simulink model "untitled"  (R2021a)
settings: Solver=VariableStepAuto  StartTime=0.0  StopTime=2  RelTol=1e-3
undefined symbols (not defined in the file or in its folder): sigbuilder_block
libraries: fuzblock x4
(part 2 of 2)

== matlab function untitled/MATLAB Function1 ==
  data: q input; C output; qd input
% Copyright (C) 2022 All rights reserved.
% Authors:     Seonghyeon Jo <cpsc.seonghyeon@gmail.com>
%
% Date:        Jan, 18, 2022
% 
% -------------------------------------------------
% Sawyer Robot 4-DoF
% get a coriolis matrix.
% -------------------------------------------------
% Equation)
%       c(q, dq)
%
% Input)
%       x   : Joint Position
%       dx  : Joint Velocity
% Output)
%       C  : Coriolis Matrix
%
% the following code has been tested on Matlab 2021a
function C = compute_C_4DOF(q,qd)
q1=q(1);
q2=q(2);
q3=q(3);
q4=q(4);
qd1=qd(1);
qd2=qd(2);
qd3=qd(3);
qd4=qd(4);
t2 = cos(q2);
t3 = sin(q2);
t4 = t3.*6.123233995736766e-17;
t5 = t2.*6.123233995736766e-17;
t6 = cos(q3);
t7 = t3-t5;
t8 = sin(q3);
t9 = t3.*3.749399456654644e-33;
t10 = t5+t9;
t11 = cos(q4);
t12 = t2+t4;
t13 = sin(q4);
t16 = t2.*3.749399456654644e-33;
t14 = t4-t16+3.749399456654644e-33;
t24 = t6.*t12;
t25 = t8.*t14;
t15 = t24-t25;
t17 = t6.*t14.*6.123233995736766e-17;
t18 = t8.*t12.*6.123233995736766e-17;
t19 = t3-t5+t17+t18-2.295845021658468e-49;
t20 = sin(q1);
t21 = cos(q1);
t23 = t21.*6.123233995736766e-17;
t22 = t20-t23;
t26 = t6.*t10.*6.123233995736766e-17;
t28 = t7.*t8.*6.123233995736766e-17;
t27 = t2+t4+t26-t28;
t29 = t6.*t7;
t30 = t8.*t10;
t31 = t29+t30;
t32 = t3.*t20.*6.123233995736766e-17;
t33 = t2.*t22;
t34 = t32+t33;
t35 = t2.*t20.*3.749399456654644e-33;
t40 = t3.*t22.*6.123233995736766e-17;
t36 = t35-t40;
t37 = t2.*t20.*6.123233995736766e-17;
t38 = t2.*(t20-t23);
t39 = t32+t38;
t41 = t6.*t36.*6.123233995736766e-17;
t42 = t6.*t39;
t43 = t8.*t36;
t44 = t42+t43;
t46 = t3.*t22;
t45 = t37-t46;
t47 = t20.*6.123233995736766e-17;
t51 = t3.*t20.*3.749399456654644e-33;
t52 = t2.*t22.*6.123233995736766e-17;
t48 = t21+t47-t51-t52;
t49 = t20.*3.749399456654644e-33;
t50 = t8.*t45.*6.123233995736766e-17;
t82 = t6.*t48.*6.123233995736766e-17;
t53 = t23+t32+t38+t49+t50-t82;
t54 = t6.*t45;
t55 = t8.*t48;
t56 = t54+t55;
t57 = t21+t47;
t58 = t2.*t21.*3.749399456654644e-33;
t68 = t3.*t57.*6.123233995736766e-17;
t59 = t58-t68;
t60 = t3.*t21.*6.123233995736766e-17;
t61 = t2.*t57;
t62 = t60+t61;
t63 = t3.*t21.*3.749399456654644e-33;
t64 = t2.*t57.*6.123233995736766e-17;
t65 = t20-t23+t63+t64;
t66 = t2.*t21.*6.123233995736766e-17;
t69 = t3.*t57;
t67 = t66-t69;
t70 = t8.*t59;
t71 = t6.*t62;
t72 = t70+t71;
t73 = t6.*t59.*6.123233995736766e-17;
t83 = t8.*t62.*6.123233995736766e-17;
t74 = t66-t69+t73-t83;
t75 = t21.*3.749399456654644e-33;
t76 = t6.*t65.*6.123233995736766e-17;
t77 = t8.*t67.*6.123233995736766e-17;
t78 = -t47+t60+t61+t75+t76+t77;
t79 = t6.*t67;
t80 = t7.*t8;
t235 = t8.*t39.*6.123233995736766e-17;
t81 = t37+t41-t46-t235;
t85 = t8.*t65;
t84 = t79-t85;
t86 = t6.*t14;
t87 = t8.*t12;
t88 = t8.*t14.*4.4101e-6;
t89 = t21.*1.925e-1;
t90 = t20.*8.100000000000001e-2;
t91 = t3.*t20.*1.688910400704115e-17;
t92 = t8.*t45.*1.4967e-2;
t93 = t2.*(t20-t23).*2.7582e-1;
t333 = t6.*t45.*1.6044e-4;
t334 = t6.*t48.*1.4967e-2;
t335 = t8.*t48.*1.6044e-4;
t94 = t89+t90+t91+t92+t93-t333-t334-t335;
t95 = t86+t87;
t96 = t2.*3.366880115214081e-34;
t97 = t11.*t15.*2.53401226709415e-4;
t98 = t6.*t14.*8.979785040610579e-2;
t99 = t8.*t12.*8.979785040610579e-2;
t201 = t3.*5.498532503507515e-18;
t202 = t13.*t15.*4.876002456295764e-2;
t203 = t11.*t19.*4.876002456295764e-2;
t204 = t13.*t19.*2.53401226709415e-4;
t100 = t96+t97+t98+t99-t201-t202-t203-t204+1.2623778474605e-66;
t101 = -t4+t16+t86+t87+1.405799628556214e-65;
t102 = t6.*t12.*6.123233995736766e-17;
t104 = t8.*t14.*6.123233995736766e-17;
t103 = t102-t104;
t105 = t21.*8.100000000000001e-2;
t106 = t3.*t21.*1.688910400704115e-17;
t107 = t6.*t65.*1.4967e-2;
t108 = t8.*t65.*1.6044e-4;
t109 = t8.*t67.*1.4967e-2;
t110 = t2.*t57.*2.7582e-1;
t282 = t20.*1.925e-1;
t283 = t6.*t67.*1.6044e-4;
t111 = t105+t106+t107+t108+t109+t110-t282-t283;
t112 = t3.*3.3204e-3;
t113 = t6.*t14.*2.53e-2;
t114 = t6.*t12.*4.4101e-6;
t115 = t8.*t12.*2.53e-2;
t116 = t2.*9.157296440624334e-22;
t117 = t6.*t14.*4.4101e-6;
t118 = t8.*t14.*2.5506e-2;
t119 = t8.*t12.*4.4101e-6;
t253 = t3.*1.4955e-5;
t254 = t6.*t12.*2.5506e-2;
t120 = t116+t117+t118+t119-t253-t254+3.433436229890238e-54;
t121 = -t3+t5+2.295845021658468e-49;
t122 = t13.*t15;
t123 = t11.*t19;
t124 = t122+t123;
t125 = t2.*4.271754237092021e-36;
t126 = t11.*t15.*8.169842925973351e-1;
t127 = t6.*t14.*1.139316919009596e-3;
t128 = t8.*t12.*1.139316919009596e-3;
t209 = t3.*6.976304090397628e-20;
t210 = t13.*t15.*2.53401226709415e-4;
t211 = t11.*t19.*2.53401226709415e-4;
t212 = t13.*t19.*8.169842925973351e-1;
t129 = t125+t126+t127+t128-t209-t210-t211-t212+1.6016513015515e-68;
t130 = t2.*2.881087492837848e-33;
t131 = t11.*t15.*1.139316919009596e-3;
t132 = t6.*t14.*7.684130555159526e-1;
t133 = t8.*t12.*7.684130555159526e-1;
t324 = t3.*4.705172944303244e-17;
t325 = t13.*t15.*8.979785040610579e-2;
t326 = t11.*t19.*8.979785040610579e-2;
t327 = t13.*t19.*1.139316919009596e-3;
t134 = t130+t131+t132+t133-t324-t325-t326-t327+1.080234788022072e-65;
t135 = t6.*t67.*6.123233995736766e-17;
t178 = t8.*t65.*6.123233995736766e-17;
t136 = t135-t178;
t137 = t6.*t65;
t138 = t8.*t67;
t139 = t137+t138;
t140 = t21.*8.100000000000001e-2;
t141 = t3.*t21.*2.449293598294706e-17;
t142 = t11.*t78.*2.152934142846781e-1;
t143 = t13.*t78.*9.274373618014111e-4;
t144 = t6.*t65.*1.097689519141626e-1;
t145 = t13.*(t79-t85).*2.152934142846781e-1;
t146 = t8.*t67.*1.097689519141626e-1;
t147 = t2.*t57.*4.0e-1;
t205 = t20.*1.925e-1;
t206 = t11.*t84.*9.274373618014111e-4;
t148 = t140+t141+t142+t143+t144+t145+t146+t147-t205-t206;
t149 = t8.*t45;
t186 = t6.*t48;
t150 = t149-t186;
t151 = t6.*t45.*6.123233995736766e-17;
t152 = t8.*t48.*6.123233995736766e-17;
t153 = t151+t152;
t154 = t21.*1.925e-1;
t155 = t20.*8.100000000000001e-2;
t156 = t3.*t20.*2.449293598294706e-17;
t157 = t8.*t45.*1.097689519141626e-1;
t158 = t2.*(t20-t23).*4.0e-1;
t159 = t11.*t53.*2.152934142846781e-1;
t160 = t13.*t53.*9.274373618014111e-4;
t161 = t13.*t56.*2.152934142846781e-1;
t207 = t11.*t56.*9.274373618014111e-4;
t208 = t6.*t48.*1.097689519141626e-1;
t162 = t154+t155+t156+t157+t158+t159+t160+t161-t207-t208;
t163 = t11.*t15;
t200 = t13.*t19;
t164 = t163-t200;
t165 = t21.*3.359125e-1;
t166 = t20.*1.41345e-1;
t167 = t3.*t20.*2.94714864922868e-17;
t168 = t8.*t45.*2.6117415e-2;
t169 = t2.*(t20-t23).*4.813059e-1;
t249 = t6.*t45.*2.799678e-4;
t250 = t6.*t48.*2.6117415e-2;
t251 = t8.*t48.*2.799678e-4;
t170 = t165+t166+t167+t168+t169-t249-t250-t251;
t171 = t21.*1.41345e-1;
t172 = t3.*t21.*2.94714864922868e-17;
t173 = t6.*t65.*2.6117415e-2;
t174 = t8.*t65.*2.799678e-4;
t175 = t8.*t67.*2.6117415e-2;
t176 = t2.*t57.*4.813059e-1;
t373 = t20.*3.359125e-1;
t374 = t6.*t67.*2.799678e-4;
t177 = t171+t172+t173+t174+t175+t176-t373-t374;
t179 = t21.*4.46715e-1;
t180 = t3.*t21.*1.350785419459531e-16;
t181 = t11.*t78.*1.18734317978;
t182 = t13.*t78.*5.114817050334782e-3;
t183 = t6.*t65.*6.053757698066069e-1;
t184 = t8.*t67.*6.053757698066069e-1;
t185 = t2.*t57.*2.206;
t187 = t21.*1.0616375;
t188 = t20.*4.46715e-1;
t189 = t3.*t20.*1.350785419459531e-16;
t190 = t8.*t45.*6.053757698066069e-1;
t191 = t2.*(t20-t23).*2.206;
t192 = t11.*t53.*1.18734317978;
t193 = t13.*t53.*5.114817050334782e-3;
t194 = t13.*t56.*1.18734317978;
t198 = t11.*t56.*5.114817050334782e-3;
t199 = t6.*t48.*6.053757698066069e-1;
t195 = t187+t188+t189+t190+t191+t192+t193+t194-t198-t199;
t196 = t13.*(t79-t85).*1.18734317978;
t293 = t20.*1.0616375;
t294 = t11.*t84.*5.114817050334782e-3;
t197 = t179+t180+t181+t182+t183+t184+t185+t196-t293-t294;
t213 = t2.*2.398599999999986e-4;
t214 = t3.*2.2398e-2;
t215 = t213+t214;
t216 = t13.*t27;
t217 = t11.*t31;
t218 = t216+t217;
t219 = t2.*t20.*7.395859701019415e-18;
t220 = t3.*t20.*8.509748831328481e-19;
t221 = t21.*1.42521e-1;
t222 = t20.*8.100000000000001e-2;
t223 = t3.*t20.*1.641700266596984e-18;
t224 = t2.*(t20-t23).*2.6811e-2;
t225 = t3.*(t20-t23).*3.0849e-3;
t1223 = t2.*t20.*1.888956455344835e-19;
t226 = t221+t222+t223+t224+t225-t1223;
t227 = t2.*6.976304090397628e-20;
t228 = t3.*4.271754237092021e-36;
t229 = t11.*t27.*2.53401226709415e-4;
t230 = t13.*t27.*8.169842925973351e-1;
t231 = t11.*t31.*8.169842925973351e-1;
t232 = t7.*t8.*1.139316919009596e-3;
t401 = t13.*t31.*2.53401226709415e-4;
t402 = t6.*t10.*1.139316919009596e-3;
t233 = t227+t228+t229+t230+t231+t232-t401-t402;
t234 = t2.*t20.*1.350785419459531e-16;
t236 = t11.*t44.*5.114817050334782e-3;
t237 = t6.*t36.*6.053757698066069e-1;
t238 = t2.*1.4613e-2;
t239 = t3.*2.398600000000009e-4;
t240 = t238+t239;
t241 = (t240.*(t3-t5))./2.0;
t399 = t2.*2.033158615944436e-19;
t242 = t88+t112+t113-t114+t115-t399-7.623123809914776e-52;
t323 = t6.*t10;
t243 = t80-t323;
t244 = t2.*t20.*1.688910400704115e-17;
t245 = t6.*t39.*1.6044e-4;
t246 = t6.*t36.*1.4967e-2;
t247 = t8.*t36.*1.6044e-4;
t385 = t8.*t39.*1.4967e-2;
t481 = t3.*t22.*2.7582e-1;
t248 = t244+t245+t246+t247-t385-t481;
t252 = (t170.*t248)./2.0;
t255 = (t120.*(t29+t30))./2.0;
t256 = t2.*t20.*1.641700266596984e-18;
t257 = t3.*t20.*1.888956455344835e-19;
t258 = t2.*(t20-t23).*3.0849e-3;
t259 = t256+t257+t258-t3.*t22.*2.6811e-2;
t260 = t21.*6.42057105e-1;
t261 = t20.*3.64905e-1;
t262 = t3.*t20.*7.395859701019415e-18;
t263 = t2.*(t20-t23).*1.20783555e-1;
t264 = t3.*(t20-t23).*1.38974745e-2;
t1228 = t2.*t20.*8.509748831328481e-19;
t265 = t260+t261+t262+t263+t264-t1228;
t266 = (t259.*t265)./2.0;
t267 = t2.*t21.*7.395859701019415e-18;
t268 = t3.*t21.*8.509748831328481e-19;
t269 = t2.*t57.*1.38974745e-2;
t1229 = t3.*t57.*1.20783555e-1;
t270 = t267+t268+t269-t1229;
t271 = t21.*8.100000000000001e-2;
t272 = t3.*t21.*1.641700266596984e-18;
t273 = t2.*t57.*2.6811e-2;
t274 = t3.*t57.*3.0849e-3;
t1230 = t20.*1.42521e-1;
t1231 = t2.*t21.*1.888956455344835e-19;
t275 = t271+t272+t273+t274-t1230-t1231;
t276 = (t270.*t275)./2.0;
t277 = t2.*t21.*2.94714864922868e-17;
t278 = t6.*t59.*2.6117415e-2;
t279 = t8.*t59.*2.799678e-4;
t280 = t6.*t62.*2.799678e-4;
t1232 = t8.*t62.*2.6117415e-2;
t1233 = t3.*t57.*4.813059e-1;
t281 = t277+t278+t279+t280-t1232-t1233;
t284 = (t111.*t281)./2.0;
t285 = t11.*t27;
t423 = t13.*t31;
t286 = t285-t423;
t287 = t2.*t21.*2.449293598294706e-17;
t288 = t6.*t59.*1.097689519141626e-1;
t289 = t13.*t74.*9.274373618014111e-4;
t290 = t11.*t72.*9.274373618014111e-4;
t291 = t11.*t74.*2.152934142846781e-1;
t389 = t13.*t72.*2.152934142846781e-1;
t390 = t8.*t62.*1.097689519141626e-1;
t469 = t3.*t57.*4.0e-1;
t292 = t287+t288+t289+t290+t291-t389-t390-t469;
t295 = t2.*t21.*1.641700266596984e-18;
t296 = t3.*t21.*1.888956455344835e-19;
t297 = t2.*t57.*3.0849e-3;
t1235 = t3.*t57.*2.6811e-2;
t298 = t295+t296+t297-t1235;
t299 = t21.*3.64905e-1;
t300 = t3.*t21.*7.395859701019415e-18;
t301 = t2.*t57.*1.20783555e-1;
t302 = t3.*t57.*1.38974745e-2;
t1236 = t20.*6.42057105e-1;
t1237 = t2.*t21.*8.509748831328481e-19;
t303 = t299+t300+t301+t302-t1236-t1237;
t304 = (t298.*t303)./2.0;
t305 = t3.*3.4179e-3;
t306 = t6.*t14.*3.3204e-3;
t307 = t6.*t12.*1.4955e-5;
t308 = t8.*t12.*3.3204e-3;
t457 = t2.*2.092860147402869e-19;
t458 = t8.*t14.*1.4955e-5;
t309 = t305+t306+t307+t308-t457-t458-7.846968699526477e-52;
t310 = (t12.*t309)./2.0;
t311 = t2.*4.705172944303244e-17;
t312 = t3.*2.881087492837848e-33;
t313 = t11.*t27.*8.979785040610579e-2;
t314 = t13.*t27.*1.139316919009596e-3;
t315 = t11.*t31.*1.139316919009596e-3;
t316 = t7.*t8.*7.684130555159526e-1;
t470 = t13.*t31.*8.979785040610579e-2;
t471 = t6.*t10.*7.684130555159526e-1;
t317 = t311+t312+t313+t314+t315+t316-t470-t471;
t318 = t2.*1.4955e-5;
t319 = t3.*9.157296440624334e-22;
t320 = t8.*(t3-t5).*4.4101e-6;
t472 = t6.*t7.*2.5506e-2;
t473 = t6.*t10.*4.4101e-6;
t474 = t8.*t10.*2.5506e-2;
t321 = t318+t319+t320-t472-t473-t474;
t322 = (t15.*t321)./2.0;
t328 = t2.*t20.*2.94714864922868e-17;
t329 = t6.*t39.*2.799678e-4;
t330 = t6.*t36.*2.6117415e-2;
t331 = t8.*t36.*2.799678e-4;
t332 = t328+t329+t330+t331-t3.*t22.*4.813059e-1-t8.*t39.*2.6117415e-2;
t336 = (t94.*t332)./2.0;
t337 = t2.*2.398600000000009e-4;
t1238 = t3.*1.4613e-2;
t338 = t337-t1238+2.282446919238515e-35;
t339 = t2.*5.498532503507515e-18;
t340 = t3.*3.366880115214081e-34;
t341 = t11.*t27.*4.876002456295764e-2;
t342 = t13.*t27.*2.53401226709415e-4;
t343 = t8.*(t3-t5).*8.979785040610579e-2;
t344 = t11.*(t29+t30).*2.53401226709415e-4;
t494 = t13.*t31.*4.876002456295764e-2;
t495 = t6.*t10.*8.979785040610579e-2;
t345 = t339+t340+t341+t342+t343+t344-t494-t495;
t346 = (t124.*t345)./2.0;
t347 = t2.*t20.*2.449293598294706e-17;
t348 = t11.*t81.*2.152934142846781e-1;
t349 = t11.*t44.*9.274373618014111e-4;
t350 = t13.*t81.*9.274373618014111e-4;
t351 = t6.*t36.*1.097689519141626e-1;
t430 = t8.*t39.*1.097689519141626e-1;
t431 = t3.*t22.*4.0e-1;
t432 = t13.*t44.*2.152934142846781e-1;
t352 = t347+t348+t349+t350+t351-t430-t431-t432;
t353 = (t195.*t352)./2.0;
t354 = t2.*t21.*1.350785419459531e-16;
t355 = t6.*t59.*6.053757698066069e-1;
t356 = t13.*t74.*5.114817050334782e-3;
t357 = t11.*t72.*5.114817050334782e-3;
t358 = t11.*t74.*1.18734317978;
t1243 = t13.*t72.*1.18734317978;
t1244 = t8.*t62.*6.053757698066069e-1;
t1245 = t3.*t57.*2.206;
t359 = t354+t355+t356+t357+t358-t1243-t1244-t1245;
t360 = (t148.*t359)./2.0;
t361 = t2.*3.3204e-3;
t362 = t3.*2.033158615944436e-19;
t363 = t6.*(t3-t5).*4.4101e-6;
t364 = t6.*t10.*2.53e-2;
t365 = t8.*t10.*4.4101e-6;
t515 = t7.*t8.*2.53e-2;
t366 = t361+t362+t363+t364+t365-t515;
t367 = (t95.*t366)./2.0;
t368 = t2.*t21.*1.688910400704115e-17;
t369 = t6.*t59.*1.4967e-2;
t370 = t8.*t59.*1.6044e-4;
t371 = t6.*t62.*1.6044e-4;
t451 = t8.*t62.*1.4967e-2;
t528 = t3.*t57.*2.7582e-1;
t372 = t368+t369+t370+t371-t451-t528;
t375 = (t177.*t372)./2.0;
t376 = t2.*3.4179e-3;
t377 = t3.*2.092860147402869e-19;
t378 = t6.*t10.*3.3204e-3;
t521 = t6.*t7.*1.4955e-5;
t522 = t7.*t8.*3.3204e-3;
t523 = t8.*t10.*1.4955e-5;
t379 = t376+t377+t378-t521-t522-t523;
t380 = t2.*2.2398e-2;
t1246 = t3.*2.398599999999986e-4;
t381 = t380-t1246+1.100898668462937e-36;
t382 = t2.*t22.*1.38974745e-2;
t383 = t219+t220+t382-t3.*t22.*1.20783555e-1;
t384 = (t226.*t383)./2.0;
t386 = t6.*t14.*2.5506e-2;
t387 = t8.*t12.*2.5506e-2;
t388 = -t88+t114+t386+t387;
t391 = t13.*t95;
t742 = t11.*t103;
t392 = t391-t742;
t393 = (t100.*t392)./2.0;
t394 = t11.*t95.*1.139316919009596e-3;
t395 = t11.*t103.*8.979785040610579e-2;
t396 = t13.*t103.*1.139316919009596e-3;
t397 = t8.*t14.*7.684130555159526e-1;
t743 = t13.*t95.*8.979785040610579e-2;
t744 = t6.*t12.*7.684130555159526e-1;
t398 = t394+t395+t396+t397-t743-t744;
t400 = (t15.*t242)./2.0;
t403 = t11.*t136.*2.152934142846781e-1;
t404 = t13.*t136.*9.274373618014111e-4;
t405 = t11.*t139.*9.274373618014111e-4;
t406 = t6.*t67.*1.097689519141626e-1;
t407 = t13.*t15.*2.152934142846781e-1;
t408 = t11.*t19.*2.152934142846781e-1;
t409 = t13.*t19.*9.274373618014111e-4;
t410 = t6.*t14.*1.097689519141626e-1;
t411 = t8.*t12.*1.097689519141626e-1;
t412 = (t95.*t120)./2.0;
t413 = t6.*t65.*1.6044e-4;
t414 = t6.*t67.*1.4967e-2;
t415 = t8.*t67.*1.6044e-4;
t854 = t8.*t65.*1.4967e-2;
t416 = t413+t414+t415-t854;
t417 = t6.*t14.*1.4967e-2;
t418 = t8.*t14.*1.6044e-4;
t419 = t8.*t12.*1.4967e-2;
t420 = t6.*t12.*2.53e-2;
t863 = t8.*t14.*2.53e-2;
t421 = t117+t119+t420-t863;
t422 = (t95.*t421)./2.0;
t424 = t11.*(t29+t30);
t425 = t216+t424;
t426 = t5+t9+t80-t323;
t427 = t23+t32+t38+t49;
t428 = t3.*2.6e-1;
t463 = t2.*1.592040838891559e-17;
t464 = t11.*t15.*9.274373618014111e-4;
t429 = t407+t408+t409+t410+t411+t428-t463-t464-5.969197056312016e-50;
t433 = t6.*t14.*1.4955e-5;
t434 = t8.*t14.*3.3204e-3;
t435 = t8.*t12.*1.4955e-5;
t884 = t6.*t12.*3.3204e-3;
t436 = t433+t434+t435-t884;
t437 = (t121.*t436)./2.0;
t438 = t11.*t95.*2.53401226709415e-4;
t439 = t11.*t103.*4.876002456295764e-2;
t440 = t13.*t103.*2.53401226709415e-4;
t441 = t8.*t14.*8.979785040610579e-2;
t745 = t13.*t95.*4.876002456295764e-2;
t746 = t6.*t12.*8.979785040610579e-2;
t442 = t438+t439+t440+t441-t745-t746;
t443 = (t124.*t442)./2.0;
t444 = -t47+t60+t61+t75;
t445 = t2.*1.3582e-1;
t446 = t3.*8.316576413009676e-18;
t447 = t6.*t10.*1.4967e-2;
t448 = t8.*t10.*1.6044e-4;
t449 = t3.*1.3582e-1;
t476 = t2.*8.316576413009676e-18;
t477 = t6.*t12.*1.6044e-4;
t450 = t417+t418+t419+t449-t476-t477-3.118216708416531e-50;
t452 = t6.*t7.*1.6044e-4;
t835 = t7.*t8.*1.4967e-2;
t453 = t445+t446+t447+t448+t452-t835;
t454 = t11.*t95;
t455 = t13.*t103;
t456 = t454+t455;
t459 = t6.*t14.*1.6044e-4;
t460 = t6.*t12.*1.4967e-2;
t461 = t8.*t12.*1.6044e-4;
t849 = t8.*t14.*1.4967e-2;
t462 = t459+t460+t461-t849;
t465 = t21.*9.748438587302075e-34;
t466 = t3.*t21.*1.592040838891559e-17;
t467 = t2.*t57.*2.6e-1;
t709 = t20.*1.592040838891559e-17;
t468 = t142+t143+t144+t145+t146-t206+t465+t466+t467-t709;
t475 = (t15.*t134)./2.0;
t478 = t21.*8.316576413009676e-18;
t479 = t20.*5.092434342028338e-34;
t480 = t3.*t20.*8.316576413009676e-18;
t482 = t2.*t22.*1.3582e-1;
t483 = t92-t333-t334-t335+t478+t479+t480+t482;
t484 = t11.*t95.*8.169842925973351e-1;
t485 = t11.*t103.*2.53401226709415e-4;
t486 = t13.*t103.*8.169842925973351e-1;
t487 = t8.*t14.*1.139316919009596e-3;
t747 = t13.*t95.*2.53401226709415e-4;
t748 = t6.*t12.*1.139316919009596e-3;
t488 = t484+t485+t486+t487-t747-t748;
t489 = t6.*t45.*1.4967e-2;
t490 = t8.*t45.*1.6044e-4;
t491 = t8.*t48.*1.4967e-2;
t492 = t489+t490+t491-t6.*t48.*1.6044e-4;
t493 = t3.*2.7582e-1;
t496 = t13.*t153.*9.274373618014111e-4;
t497 = t6.*t45.*1.097689519141626e-1;
t498 = t11.*t150.*9.274373618014111e-4;
t499 = t8.*t48.*1.097689519141626e-1;
t500 = t11.*t153.*2.152934142846781e-1;
t501 = t496+t497+t498+t499+t500-t13.*t150.*2.152934142846781e-1;
t502 = t3.*4.0e-1;
t503 = t2.*2.6e-1;
t504 = t3.*1.592040838891559e-17;
t505 = t11.*t27.*2.152934142846781e-1;
t506 = t13.*t27.*9.274373618014111e-4;
t507 = t6.*t10.*1.097689519141626e-1;
t508 = t21.*1.592040838891559e-17;
t509 = t20.*9.748438587302075e-34;
t510 = t3.*t20.*1.592040838891559e-17;
t511 = t2.*t22.*2.6e-1;
t512 = t157+t159+t160+t161-t207-t208+t508+t509+t510+t511;
t513 = t11.*t31.*9.274373618014111e-4;
t594 = t13.*t31.*2.152934142846781e-1;
t845 = t7.*t8.*1.097689519141626e-1;
t514 = t503+t504+t505+t506+t507+t513-t594-t845;
t516 = t11.*t95.*9.274373618014111e-4;
t517 = t11.*t103.*2.152934142846781e-1;
t518 = t13.*t103.*9.274373618014111e-4;
t519 = t6.*t12.*1.097689519141626e-1;
t704 = t13.*t95.*2.152934142846781e-1;
t886 = t8.*t14.*1.097689519141626e-1;
t520 = t516+t517+t518+t519-t704-t886;
t524 = t21.*5.092434342028338e-34;
t525 = t3.*t21.*8.316576413009676e-18;
t526 = t2.*t57.*1.3582e-1;
t900 = t20.*8.316576413009676e-18;
t527 = t107+t108+t109-t283+t524+t525+t526-t900;
t529 = t8.*(t3-t5);
t530 = t5+t9-t323+t529;
t531 = t2.*t20.*4.271754237092021e-36;
t532 = t8.*t39.*1.139316919009596e-3;
t533 = t11.*t81.*2.53401226709415e-4;
t534 = t11.*t44.*8.169842925973351e-1;
t535 = t13.*t81.*8.169842925973351e-1;
t536 = t531+t532+t533+t534+t535-t3.*t22.*6.976304090397628e-20-t6.*t36.*1.139316919009596e-3-t13.*t44.*2.53401226709415e-4;
t537 = t21.*3.366880115214081e-34;
t538 = t20.*2.061619478104898e-50;
t539 = t3.*t20.*3.366880115214081e-34;
t540 = t2.*(t20-t23).*5.498532503507515e-18;
t541 = t11.*t53.*4.876002456295764e-2;
t542 = t13.*t53.*2.53401226709415e-4;
t543 = t13.*t56.*4.876002456295764e-2;
t544 = t6.*t48.*8.979785040610579e-2;
t685 = t8.*t45.*8.979785040610579e-2;
t686 = t11.*t56.*2.53401226709415e-4;
t545 = t537+t538+t539+t540+t541+t542+t543+t544-t685-t686;
t546 = t286.*t545;
t547 = t21.*4.271754237092021e-36;
t548 = t20.*2.615695076599444e-52;
t549 = t3.*t20.*4.271754237092021e-36;
t550 = t2.*(t20-t23).*6.976304090397628e-20;
t551 = t11.*t53.*2.53401226709415e-4;
t552 = t13.*t53.*8.169842925973351e-1;
t553 = t13.*t56.*2.53401226709415e-4;
t554 = t6.*t48.*1.139316919009596e-3;
t687 = t8.*t45.*1.139316919009596e-3;
t688 = t11.*t56.*8.169842925973351e-1;
t555 = t547+t548+t549+t550+t551+t552+t553+t554-t687-t688;
t556 = t425.*t555;
t557 = t21.*2.881087492837848e-33;
t558 = t20.*1.764157288083672e-49;
t559 = t3.*t20.*2.881087492837848e-33;
t560 = t2.*(t20-t23).*4.705172944303244e-17;
t561 = t11.*t53.*8.979785040610579e-2;
t562 = t13.*t53.*1.139316919009596e-3;
t563 = t13.*t56.*8.979785040610579e-2;
t564 = t6.*t48.*7.684130555159526e-1;
t683 = t8.*t45.*7.684130555159526e-1;
t684 = t11.*t56.*1.139316919009596e-3;
t565 = t557+t558+t559+t560+t561+t562+t563+t564-t683-t684;
t566 = t530.*t565;
t567 = t2.*t20.*2.881087492837848e-33;
t568 = t8.*t39.*7.684130555159526e-1;
t569 = t11.*t81.*8.979785040610579e-2;
t570 = t11.*t44.*1.139316919009596e-3;
t571 = t13.*t81.*1.139316919009596e-3;
t572 = t567+t568+t569+t570+t571-t3.*t22.*4.705172944303244e-17-t6.*t36.*7.684130555159526e-1-t13.*t44.*8.979785040610579e-2;
t573 = t2.*t20.*3.366880115214081e-34;
t574 = t8.*t39.*8.979785040610579e-2;
t575 = t11.*t81.*4.876002456295764e-2;
t576 = t11.*t44.*2.53401226709415e-4;
t577 = t13.*t81.*2.53401226709415e-4;
t578 = t573+t574+t575+t576+t577-t3.*t22.*5.498532503507515e-18-t6.*t36.*8.979785040610579e-2-t13.*t44.*4.876002456295764e-2;
t579 = t124.*t578;
t580 = t546+t556+t566+t579-t101.*t572-t164.*t536;
t581 = t11.*t78.*9.274373618014111e-4;
t582 = t11.*t84.*2.152934142846781e-1;
t583 = t13.*t84.*9.274373618014111e-4;
t584 = t21.*1.804275904458619e-49;
t585 = t3.*t21.*5.06463411777858e-49;
t701 = t2.*2.449293598294706e-17;
t586 = t407+t408+t409+t410+t411-t464+t502-t701-5.342894225732869e-34;
t587 = t11.*t78.*4.451823873129729e-33;
t588 = t13.*t78.*1.917749226941314e-35;
t589 = t6.*t65.*2.269795582384779e-33;
t590 = t13.*(t79-t85).*4.451823873129729e-33;
t591 = t8.*t67.*2.269795582384779e-33;
t592 = t2.*t57.*8.271175201380145e-33;
t712 = t13.*t78.*2.152934142846781e-1;
t593 = t581+t582+t583-t712;
t595 = t11.*t15.*8.979785040610579e-2;
t596 = t13.*t15.*1.139316919009596e-3;
t597 = t11.*t19.*1.139316919009596e-3;
t749 = t13.*t19.*8.979785040610579e-2;
t598 = t595+t596+t597-t749;
t599 = t20.*2.295845021658468e-49;
t600 = t2.*2.540928714850161e-34;
t601 = t6.*t14.*6.776895191416263e-2;
t602 = t8.*t12.*6.776895191416263e-2;
t641 = t3.*4.149651502162508e-18;
t603 = t407+t408+t409-t464+t600+t601+t602-t641+9.526956742857376e-67;
t604 = t21.*2.540928714850161e-34;
t605 = t20.*1.555870108751424e-50;
t606 = t3.*t20.*2.540928714850161e-34;
t607 = t2.*(t20-t23).*4.149651502162508e-18;
t608 = t6.*t48.*6.776895191416263e-2;
t609 = -t159-t160-t161+t207+t604+t605+t606+t607+t608-t8.*t45.*6.776895191416263e-2;
t610 = t51+t52+t75-t149+t186+t599;
t611 = t13.*t15.*8.169842925973351e-1;
t612 = t11.*t19.*8.169842925973351e-1;
t613 = t97-t204+t611+t612;
t614 = t21.*2.061619478104898e-50;
t615 = t3.*t21.*3.366880115214081e-34;
t616 = t11.*t78.*4.876002456295764e-2;
t617 = t13.*t78.*2.53401226709415e-4;
t618 = t2.*t57.*5.498532503507515e-18;
t619 = t13.*t84.*4.876002456295764e-2;
t668 = t20.*3.366880115214081e-34;
t669 = t6.*t65.*8.979785040610579e-2;
t670 = t11.*t84.*2.53401226709415e-4;
t671 = t8.*t67.*8.979785040610579e-2;
t620 = t614+t615+t616+t617+t618+t619-t668-t669-t670-t671;
t621 = t21.*2.615695076599444e-52;
t622 = t3.*t21.*4.271754237092021e-36;
t623 = t11.*t78.*2.53401226709415e-4;
t624 = t13.*t78.*8.169842925973351e-1;
t625 = t2.*t57.*6.976304090397628e-20;
t626 = t21.*1.764157288083672e-49;
t627 = t3.*t21.*2.881087492837848e-33;
t628 = t11.*t78.*8.979785040610579e-2;
t629 = t13.*t78.*1.139316919009596e-3;
t630 = t2.*t57.*4.705172944303244e-17;
t631 = t8.*(t3-t5).*1.139316919009596e-3;
t632 = t11.*(t29+t30).*8.169842925973351e-1;
t633 = t227+t228+t229+t230-t401-t402+t631+t632;
t634 = t8.*(t3-t5).*7.684130555159526e-1;
t635 = t11.*(t29+t30).*1.139316919009596e-3;
t636 = t311+t312+t313+t314-t470-t471+t634+t635;
t637 = t11.*t15.*2.152934142846781e-1;
t638 = t13.*t15.*9.274373618014111e-4;
t639 = t11.*t19.*9.274373618014111e-4;
t720 = t13.*t19.*2.152934142846781e-1;
t640 = t637+t638+t639-t720;
t642 = t21.*2.295845021658468e-49;
t643 = t2.*4.149651502162508e-18;
t644 = t3.*2.540928714850161e-34;
t645 = t6.*t10.*6.776895191416263e-2;
t646 = t49-t63-t64+t137+t138-t642;
t1187 = t7.*t8.*6.776895191416263e-2;
t647 = t505+t506+t513-t594-t643-t644+t645-t1187;
t648 = t20.*2.540928714850161e-34;
t649 = t6.*t65.*6.776895191416263e-2;
t650 = t8.*t67.*6.776895191416263e-2;
t705 = t21.*1.555870108751424e-50;
t706 = t3.*t21.*2.540928714850161e-34;
t707 = t2.*t57.*4.149651502162508e-18;
t651 = t142+t143+t145-t206+t648+t649+t650-t705-t706-t707;
t652 = t11.*t15.*4.876002456295764e-2;
t821 = t13.*t19.*4.876002456295764e-2;
t653 = t210+t211+t652-t821;
t654 = (t124.*t653)./2.0;
t655 = t2.*t21.*3.366880115214081e-34;
t656 = t13.*t74.*2.53401226709415e-4;
t657 = t11.*t72.*2.53401226709415e-4;
t658 = t8.*t62.*8.979785040610579e-2;
t659 = t11.*t74.*4.876002456295764e-2;
t864 = t6.*t59.*8.979785040610579e-2;
t865 = t13.*t72.*4.876002456295764e-2;
t866 = t3.*t57.*5.498532503507515e-18;
t660 = t655+t656+t657+t658+t659-t864-t865-t866;
t661 = t124.*t660;
t662 = t2.*t21.*4.271754237092021e-36;
t663 = t13.*t74.*8.169842925973351e-1;
t664 = t11.*t72.*8.169842925973351e-1;
t665 = t8.*t62.*1.139316919009596e-3;
t666 = t11.*t74.*2.53401226709415e-4;
t867 = t6.*t59.*1.139316919009596e-3;
t868 = t13.*t72.*2.53401226709415e-4;
t869 = t3.*t57.*6.976304090397628e-20;
t667 = t662+t663+t664+t665+t666-t867-t868-t869;
t672 = t13.*(t79-t85).*2.53401226709415e-4;
t715 = t20.*4.271754237092021e-36;
t716 = t6.*t65.*1.139316919009596e-3;
t717 = t11.*t84.*8.169842925973351e-1;
t718 = t8.*t67.*1.139316919009596e-3;
t673 = t621+t622+t623+t624+t625+t672-t715-t716-t717-t718;
t674 = t13.*(t79-t85).*8.979785040610579e-2;
t737 = t20.*2.881087492837848e-33;
t738 = t6.*t65.*7.684130555159526e-1;
t739 = t11.*t84.*1.139316919009596e-3;
t740 = t8.*t67.*7.684130555159526e-1;
t675 = t626+t627+t628+t629+t630+t674-t737-t738-t739-t740;
t676 = t2.*t21.*2.881087492837848e-33;
t677 = t13.*t74.*1.139316919009596e-3;
t678 = t11.*t72.*1.139316919009596e-3;
t679 = t8.*t62.*7.684130555159526e-1;
t680 = t11.*t74.*8.979785040610579e-2;
t872 = t6.*t59.*7.684130555159526e-1;
t873 = t13.*t72.*8.979785040610579e-2;
t874 = t3.*t57.*4.705172944303244e-17;
t681 = t676+t677+t678+t679+t680-t872-t873-t874;
t682 = t286.*t620;
t689 = t11.*t53.*9.274373618014111e-4;
t690 = t11.*t56.*2.152934142846781e-1;
t691 = t13.*t56.*9.274373618014111e-4;
t692 = t689+t690+t691-t13.*t53.*2.152934142846781e-1;
t693 = t21.*2.946606165491677e-33;
t694 = t20.*1.804275904458619e-49;
t695 = t3.*t20.*5.06463411777858e-49;
t696 = t8.*t45.*2.269795582384779e-33;
t697 = t2.*(t20-t23).*8.271175201380145e-33;
t698 = t11.*t53.*4.451823873129729e-33;
t699 = t13.*t53.*1.917749226941314e-35;
t700 = t13.*t56.*4.451823873129729e-33;
t702 = t57.*t586.*5.515;
t703 = t693+t694+t695+t696+t697+t698+t699+t700+t702-t6.*t48.*2.269795582384779e-33-t11.*t56.*1.917749226941314e-35;
t708 = t429.*t444.*5.515;
t710 = t121.*t468.*5.515;
t711 = t708+t710;
t713 = t101.*t651.*5.515;
t1063 = t603.*t646.*5.515;
t714 = t713-t1063;
t719 = t13.*t84.*2.53401226709415e-4;
t721 = t2.*(t20-t23).*6.123233995736766e-17;
t722 = t51+t75-t149+t186+t599+t721;
t723 = t11.*t53;
t724 = t13.*t56;
t725 = t723+t724;
t726 = t13.*t53;
t727 = -t20+t23;
t728 = t3.*t727;
t729 = t37+t728;
t730 = t2.*t727.*6.123233995736766e-17;
t731 = t21+t47-t51+t730;
t732 = t6.*t729;
t733 = t8.*t731;
t734 = t732+t733;
t735 = t8.*t729.*6.123233995736766e-17;
t752 = t2.*t727;
t753 = t6.*t731.*6.123233995736766e-17;
t736 = t23+t32+t49+t735-t752-t753;
t741 = t726-t11.*t56;
t750 = t6.*t731;
t754 = t8.*t729;
t751 = t51+t75+t599-t730+t750-t754;
t755 = t6.*t729.*6.123233995736766e-17;
t756 = t8.*t731.*6.123233995736766e-17;
t757 = t755+t756;
t758 = t750-t754;
t759 = t11.*t734.*9.274373618014111e-4;
t760 = t11.*t736;
t761 = t13.*t734;
t762 = t760+t761;
t763 = t13.*(t79-t85).*4.876002456295764e-2;
t764 = t614+t615+t616+t617+t618-t668-t669-t670-t671+t763;
t765 = t11.*t734;
t797 = t13.*t736;
t766 = t765-t797;
t767 = t675.*t751;
t768 = t11.*t736.*8.979785040610579e-2;
t769 = t13.*t736.*1.139316919009596e-3;
t770 = t13.*t734.*8.979785040610579e-2;
t771 = t6.*t731.*7.684130555159526e-1;
t790 = t8.*t729.*7.684130555159526e-1;
t791 = t2.*t727.*4.705172944303244e-17;
t792 = t11.*t734.*1.139316919009596e-3;
t772 = t557+t558+t559+t768+t769+t770+t771-t790-t791-t792;
t773 = t11.*t78;
t774 = t13.*(t79-t85);
t775 = t773+t774;
t776 = t11.*t736.*4.876002456295764e-2;
t777 = t13.*t736.*2.53401226709415e-4;
t778 = t13.*t734.*4.876002456295764e-2;
t779 = t6.*t731.*8.979785040610579e-2;
t794 = t8.*t729.*8.979785040610579e-2;
t795 = t2.*t727.*5.498532503507515e-18;
t796 = t11.*t734.*2.53401226709415e-4;
t780 = t537+t538+t539+t776+t777+t778+t779-t794-t795-t796;
t781 = t775.*t780;
t782 = t13.*t78;
t793 = t11.*t84;
t783 = t782-t793;
t784 = t11.*t736.*2.53401226709415e-4;
t785 = t13.*t736.*8.169842925973351e-1;
t786 = t13.*t734.*2.53401226709415e-4;
t787 = t6.*t731.*1.139316919009596e-3;
t798 = t8.*t729.*1.139316919009596e-3;
t799 = t2.*t727.*6.976304090397628e-20;
t800 = t11.*t734.*8.169842925973351e-1;
t788 = t547+t548+t549+t784+t785+t786+t787-t798-t799-t800;
t789 = t783.*t788;
t801 = t646.*t675;
t802 = t11.*t736.*9.274373618014111e-4;
t803 = t11.*t734.*2.152934142846781e-1;
t804 = t13.*t734.*9.274373618014111e-4;
t1111 = t13.*t736.*2.152934142846781e-1;
t805 = t802+t803+t804-t1111;
t806 = t23+t32+t49-t752;
t807 = t8.*t729.*1.097689519141626e-1;
t808 = t11.*t736.*2.152934142846781e-1;
t809 = t13.*t736.*9.274373618014111e-4;
t810 = t13.*t734.*2.152934142846781e-1;
t811 = t764.*t775;
t812 = t673.*t783;
t813 = -t801+t811+t812;
t819 = t646.*t772;
t814 = t781+t789-t819;
t815 = t751.*t772;
t816 = t762.*t780;
t817 = t762.*t764;
t818 = t129.*t783.*3.749399456654644e-33;
t820 = t100.*t775.*3.749399456654644e-33;
t822 = t6.*t12.*6.776895191416263e-2;
t1058 = t8.*t14.*6.776895191416263e-2;
t823 = t516+t517+t518-t704+t822-t1058;
t824 = t6.*t731.*6.776895191416263e-2;
t825 = t13.*t757.*9.274373618014111e-4;
t826 = t11.*t757.*2.152934142846781e-1;
t830 = t6.*t731.*1.097689519141626e-1;
t888 = t2.*t727.*4.0e-1;
t827 = t154+t155+t156-t759+t807+t808+t809+t810-t830-t888;
t828 = t13.*t758.*2.152934142846781e-1;
t833 = t13.*t139.*2.152934142846781e-1;
t853 = t8.*t65.*1.097689519141626e-1;
t829 = t403+t404+t405+t406-t833-t853;
t1032 = t766.*t788;
t831 = t801-t811-t812+t815+t816-t1032;
t1028 = t673.*t766;
t832 = t767+t781+t789+t817-t819-t1028;
t1107 = t8.*t729.*6.776895191416263e-2;
t1108 = t2.*t727.*4.149651502162508e-18;
t834 = t604+t605+t606+t759-t808-t809-t810+t824-t1107-t1108;
t836 = t2.*t20.*8.316576413009676e-18;
t837 = t32-t752;
t838 = t3.*t727.*6.123233995736766e-17;
t839 = t35+t838;
t840 = t8.*t729.*1.4967e-2;
t841 = t2.*t21.*1.592040838891559e-17;
t1359 = t3.*t57.*2.6e-1;
t842 = t288+t289+t290+t291-t389-t390+t841-t1359;
t843 = t121.*t842.*5.515;
t844 = t67.*t429.*5.515;
t846 = t444.*t514.*5.515;
t1560 = t12.*t468.*5.515;
t847 = t843+t844+t846-t1560;
t848 = t129.*t425.*1.874699728327322e-33;
t850 = t57.*t462.*(3.49e2./2.0e2);
t911 = t6.*t729.*1.6044e-4;
t912 = t6.*t731.*1.4967e-2;
t913 = t8.*t731.*1.6044e-4;
t979 = t2.*t727.*2.7582e-1;
t851 = t89+t90+t91+t840-t911-t912-t913-t979;
t852 = t164.*t633.*1.874699728327322e-33;
t855 = t21.*5.708905626981487e-50;
t856 = t3.*t21.*1.105003754409848e-49;
t857 = t6.*t65.*9.792462161022385e-35;
t858 = t8.*t65.*1.049711117200796e-36;
t919 = t2.*1.688910400704115e-17;
t859 = t417+t418+t419-t477+t493-t919-5.342894225732868e-34;
t860 = t8.*t67.*9.792462161022385e-35;
t861 = t2.*t57.*1.804608079944675e-33;
t862 = t242.*(t80-t323).*1.874699728327322e-33;
t870 = t425.*t673;
t871 = t530.*t675;
t875 = t429.*t806.*5.515;
t968 = t2.*t727.*2.6e-1;
t876 = t508+t509+t510-t759+t807+t808+t809+t810-t830-t968;
t877 = t121.*t876.*5.515;
t878 = t875+t877;
t879 = t6.*t839.*6.123233995736766e-17;
t963 = t8.*t837.*6.123233995736766e-17;
t880 = t37+t728+t879-t963;
t881 = t6.*t837;
t882 = t8.*t839;
t883 = t881+t882;
t885 = t100.*t286.*1.874699728327322e-33;
t887 = t57.*t520.*5.515;
t889 = t21.*9.157296440624334e-22;
t890 = t20.*5.60722688742702e-38;
t891 = t3.*t20.*9.157296440624334e-22;
t892 = t21.*2.033158615944436e-19;
t893 = t20.*1.244950595587608e-35;
t894 = t3.*t20.*2.033158615944436e-19;
t895 = t21.*2.092860147402869e-19;
t896 = t20.*1.281507240289991e-35;
t897 = t3.*t20.*2.092860147402869e-19;
t898 = t2.*t20.*2.033158615944436e-19;
t899 = t67.*t450.*(3.49e2./2.0e2);
t901 = t2.*t21.*8.316576413009676e-18;
t1350 = t3.*t57.*1.3582e-1;
t902 = t369+t370+t371-t451+t901-t1350;
t903 = t121.*t902.*(3.49e2./2.0e2);
t904 = t444.*t453.*(3.49e2./2.0e2);
t1425 = t12.*t527.*(3.49e2./2.0e2);
t905 = t899+t903+t904-t1425;
t906 = t6.*t65.*1.049711117200796e-36;
t907 = t6.*t67.*9.792462161022385e-35;
t908 = t8.*t67.*1.049711117200796e-36;
t909 = t101.*t636.*1.874699728327322e-33;
t910 = t134.*t530.*1.874699728327322e-33;
t914 = t6.*t837.*1.6044e-4;
t915 = t6.*t839.*1.4967e-2;
t916 = t8.*t839.*1.6044e-4;
t917 = t21.*9.323350423903855e-34;
t918 = t20.*5.708905626981487e-50;
t920 = t57.*t859.*(3.49e2./2.0e2);
t921 = t3.*t20.*1.105003754409848e-49;
t922 = t6.*t729.*1.097689519141626e-1;
t923 = t8.*t731.*1.097689519141626e-1;
t924 = t21.*1.244950595587608e-35;
t925 = t3.*t21.*2.033158615944436e-19;
t926 = t6.*t65.*2.53e-2;
t927 = t8.*t65.*4.4101e-6;
t928 = t8.*t67.*2.53e-2;
t929 = t2.*t57.*3.3204e-3;
t1005 = t20.*2.033158615944436e-19;
t1006 = t6.*t67.*4.4101e-6;
t930 = t924+t925+t926+t927+t928+t929-t1005-t1006;
t931 = t6.*t59.*4.4101e-6;
t932 = t8.*t59.*2.5506e-2;
t933 = t6.*t62.*2.5506e-2;
t934 = t3.*t57.*1.4955e-5;
t1523 = t2.*t21.*9.157296440624334e-22;
t1524 = t8.*t62.*4.4101e-6;
t935 = t931+t932+t933+t934-t1523-t1524;
t936 = t21.*1.281507240289991e-35;
t937 = t3.*t21.*2.092860147402869e-19;
t938 = t6.*t65.*3.3204e-3;
t939 = t6.*t67.*1.4955e-5;
t940 = t8.*t67.*3.3204e-3;
t941 = t2.*t57.*3.4179e-3;
t1013 = t20.*2.092860147402869e-19;
t1014 = t8.*t65.*1.4955e-5;
t942 = t936+t937+t938+t939+t940+t941-t1013-t1014;
t943 = t12.*t942;
t944 = t2.*t21.*2.033158615944436e-19;
t945 = t6.*t59.*2.53e-2;
t946 = t8.*t59.*4.4101e-6;
t947 = t6.*t62.*4.4101e-6;
t1526 = t8.*t62.*2.53e-2;
t1527 = t3.*t57.*3.3204e-3;
t948 = t944+t945+t946+t947-t1526-t1527;
t949 = t95.*t948;
t950 = t8.*t59.*1.4955e-5;
t951 = t6.*t62.*1.4955e-5;
t952 = t8.*t62.*3.3204e-3;
t953 = t3.*t57.*3.4179e-3;
t1528 = t2.*t21.*2.092860147402869e-19;
t1529 = t6.*t59.*3.3204e-3;
t954 = t950+t951+t952+t953-t1528-t1529;
t955 = t121.*t954;
t956 = t20.*9.157296440624334e-22;
t957 = t3.*t21.*9.157296440624334e-22;
t958 = t6.*t67.*2.5506e-2;
t959 = t2.*t57.*1.4955e-5;
t997 = t21.*5.60722688742702e-38;
t998 = t6.*t65.*4.4101e-6;
t999 = t8.*t65.*2.5506e-2;
t1000 = t8.*t67.*4.4101e-6;
t960 = -t956+t957+t958+t959+t997-t998-t999-t1000;
t1522 = t243.*t930;
t1525 = t15.*t935;
t1530 = t31.*t960;
t961 = t943+t949+t955-t1522-t1525-t1530;
t962 = t2.*t20.*1.592040838891559e-17;
t964 = t11.*t880.*2.152934142846781e-1;
t965 = t11.*t883.*9.274373618014111e-4;
t966 = t13.*t880.*9.274373618014111e-4;
t967 = t6.*t839.*1.097689519141626e-1;
t969 = t11.*t136.*4.451823873129729e-33;
t970 = t13.*t136.*1.917749226941314e-35;
t971 = t11.*t139.*1.917749226941314e-35;
t972 = t6.*t67.*2.269795582384779e-33;
t973 = t121.*t379.*1.874699728327322e-33;
t974 = t444.*t450.*(3.49e2./2.0e2);
t975 = t121.*t527.*(3.49e2./2.0e2);
t976 = t974+t975;
t995 = t11.*t758.*9.274373618014111e-4;
t977 = t825+t826+t828+t922+t923-t995;
t1322 = t2.*t727.*1.3582e-1;
t978 = t478+t479+t480+t840-t911-t912-t913-t1322;
t980 = t6.*t65.*2.799678e-4;
t981 = t6.*t67.*2.6117415e-2;
t982 = t8.*t67.*2.799678e-4;
t1361 = t8.*t65.*2.6117415e-2;
t983 = t980+t981+t982-t1361;
t984 = (t111.*t983)./2.0;
t985 = t11.*t136.*1.18734317978;
t986 = t13.*t136.*5.114817050334782e-3;
t987 = t11.*t139.*5.114817050334782e-3;
t988 = t6.*t67.*6.053757698066069e-1;
t1351 = t8.*t65.*6.053757698066069e-1;
t1352 = t13.*t139.*1.18734317978;
t2028 = t985+t986+t987+t988-t1351-t1352;
t989 = (t148.*t2028)./2.0;
t990 = t6.*t729.*1.4967e-2;
t991 = t8.*t729.*1.6044e-4;
t992 = t8.*t731.*1.4967e-2;
t1370 = t6.*t731.*1.6044e-4;
t993 = t990+t991+t992-t1370;
t994 = (t177.*t416)./2.0;
t996 = (t197.*t829)./2.0;
t1001 = t6.*t729.*2.5506e-2;
t1002 = t6.*t731.*4.4101e-6;
t1003 = t8.*t731.*2.5506e-2;
t1017 = t8.*t729.*4.4101e-6;
t1018 = t2.*t727.*1.4955e-5;
t1004 = t889+t890+t891+t1001+t1002+t1003-t1017-t1018;
t1007 = t8.*t729.*2.53e-2;
t1019 = t6.*t729.*4.4101e-6;
t1020 = t2.*t727.*3.3204e-3;
t1021 = t6.*t731.*2.53e-2;
t1022 = t8.*t731.*4.4101e-6;
t1008 = t892+t893+t894+t1007-t1019-t1020-t1021-t1022;
t1009 = t6.*t729.*1.4955e-5;
t1010 = t8.*t729.*3.3204e-3;
t1011 = t8.*t731.*1.4955e-5;
t1015 = t2.*t727.*3.4179e-3;
t1016 = t6.*t731.*3.3204e-3;
t1012 = t895+t896+t897+t1009+t1010+t1011-t1015-t1016;
t1023 = t444.*t1012;
t1024 = t1004.*(t79-t85);
t1025 = t139.*t1008;
t1026 = t139.*t930;
t1027 = t444.*t942;
t1029 = t727.*t832;
t1030 = t100.*t762.*3.749399456654644e-33;
t1031 = t134.*t751.*3.749399456654644e-33;
t1033 = t57.*t813;
t1034 = t727.*t813;
t1035 = t57.*t814;
t1038 = t134.*t646.*3.749399456654644e-33;
t1036 = t818+t820+t1034+t1035-t1038;
t1037 = t57.*t832;
t1039 = t242.*(t750-t754).*3.749399456654644e-33;
t1040 = t120.*t734.*3.749399456654644e-33;
t1041 = t734.*t960;
t1042 = t806.*t942;
t1043 = t758.*t1008;
t1044 = t960.*(t79-t85);
t1045 = t1026+t1027+t1044;
t1046 = t1023+t1024+t1025;
t1047 = t815+t816-t1032;
t1048 = t767+t817-t1028;
t1049 = t734.*t1004;
t1050 = t806.*t1012;
t1051 = -t1043+t1049+t1050;
t1053 = t758.*t930;
t1052 = t1041+t1042-t1053;
t1054 = t84.*t960;
t1055 = t84.*t120.*3.749399456654644e-33;
t1056 = t6.*t67.*6.776895191416263e-2;
t1851 = t8.*t65.*6.776895191416263e-2;
t1852 = t403+t404+t405-t833+t1056-t1851;
t1057 = t101.*t1852.*5.515;
t1059 = t15.*t651.*5.515;
t1898 = t84.*t603.*5.515;
t1899 = t646.*t823.*5.515;
t1060 = t1057+t1059-t1898-t1899;
t1061 = (t148.*t1060)./2.0;
t1062 = t100.*t164.*1.874699728327322e-33;
t1064 = t11.*t78.*1.139316919009596e-3;
t1065 = t11.*t84.*8.979785040610579e-2;
t1066 = t13.*t84.*1.139316919009596e-3;
t1824 = t13.*t78.*8.979785040610579e-2;
t1067 = t1064+t1065+t1066-t1824;
t1068 = t11.*t78.*8.169842925973351e-1;
t1069 = t13.*t84.*8.169842925973351e-1;
t1070 = -t617+t670+t1068+t1069;
t1071 = t124.*t673;
t1072 = t11.*t84.*4.876002456295764e-2;
t1826 = t13.*t78.*4.876002456295764e-2;
t1073 = t124.*(t623+t719+t1072-t1826);
t1074 = t100.*t762;
t1075 = t134.*t751;
t1142 = t129.*t766;
t1076 = t1074+t1075-t1142;
t1077 = t121.*t1076;
t1078 = t121.*t593.*5.515;
t1079 = t444.*t640.*5.515;
t1080 = t1078+t1079;
t1081 = t100.*t392;
t1082 = t124.*t442;
t1083 = t15.*t134;
t1829 = t101.*t398;
t1830 = t129.*t456;
t1831 = t164.*t488;
t1084 = t1081+t1082+t1083-t1829-t1830-t1831;
t1085 = (t121.*t1084)./2.0;
t1086 = t101.*t598.*1.874699728327322e-33;
t1087 = t164.*t613.*1.874699728327322e-33;
t1088 = t392.*t764;
t1089 = t11.*t136.*4.876002456295764e-2;
t1090 = t13.*t136.*2.53401226709415e-4;
t1091 = t8.*t65.*8.979785040610579e-2;
t1092 = t11.*t139.*2.53401226709415e-4;
t1859 = t6.*t67.*8.979785040610579e-2;
t1860 = t13.*t139.*4.876002456295764e-2;
t1093 = t1089+t1090+t1091+t1092-t1859-t1860;
t1094 = t11.*t136.*2.53401226709415e-4;
t1095 = t13.*t136.*8.169842925973351e-1;
t1096 = t8.*t65.*1.139316919009596e-3;
t1097 = t11.*t139.*8.169842925973351e-1;
t1862 = t6.*t67.*1.139316919009596e-3;
t1863 = t13.*t139.*2.53401226709415e-4;
t2210 = t1094+t1095+t1096+t1097-t1862-t1863;
t1098 = t164.*t2210;
t1099 = t15.*t675;
t1100 = t11.*t136.*8.979785040610579e-2;
t1101 = t13.*t136.*1.139316919009596e-3;
t1102 = t8.*t65.*7.684130555159526e-1;
t1103 = t11.*t139.*1.139316919009596e-3;
t1864 = t6.*t67.*7.684130555159526e-1;
t1865 = t13.*t139.*8.979785040610579e-2;
t2207 = t1100+t1101+t1102+t1103-t1864-t1865;
t1104 = t101.*t2207;
t1858 = t456.*t673;
t1861 = t124.*t1093;
t1105 = t1088+t1098+t1099+t1104-t1858-t1861;
t1106 = (t444.*t1105)./2.0;
t1109 = t101.*t834.*5.515;
t1188 = t603.*t751.*5.515;
t1110 = t1109-t1188;
t1112 = t124.*t129.*1.874699728327322e-33;
t1113 = t121.*t805.*5.515;
t1114 = t640.*t806.*5.515;
t1115 = t1113+t1114;
t1116 = t129.*t783;
t1117 = t100.*t775;
t1138 = t134.*t646;
t1118 = t1116+t1117-t1138;
t1119 = t121.*t1118;
t1120 = t603.*t734.*5.515;
t1121 = t15.*t834.*5.515;
t1122 = t6.*t729.*6.776895191416263e-2;
t1123 = t8.*t731.*6.776895191416263e-2;
t1124 = t6.*t729.*7.684130555159526e-1;
t1125 = t11.*t758.*1.139316919009596e-3;
t1126 = t8.*t731.*7.684130555159526e-1;
t1900 = t13.*t757.*1.139316919009596e-3;
t1901 = t11.*t757.*8.979785040610579e-2;
t1902 = t13.*t758.*8.979785040610579e-2;
t1127 = t1124+t1125+t1126-t1900-t1901-t1902;
t1128 = t15.*t772;
t1129 = t6.*t729.*8.979785040610579e-2;
t1130 = t11.*t758.*2.53401226709415e-4;
t1131 = t8.*t731.*8.979785040610579e-2;
t1132 = t392.*t780;
t1133 = t6.*t729.*1.139316919009596e-3;
t1134 = t11.*t758.*8.169842925973351e-1;
t1135 = t8.*t731.*1.139316919009596e-3;
t1904 = t13.*t757.*8.169842925973351e-1;
t1905 = t11.*t757.*2.53401226709415e-4;
t1906 = t13.*t758.*2.53401226709415e-4;
t1136 = t1133+t1134+t1135-t1904-t1905-t1906;
t1137 = t444.*t813;
t1139 = t806.*t814;
t1140 = t1119+t1137+t1139;
t1141 = t444.*t1048;
t1143 = t806.*t1047;
t1144 = t1077+t1141+t1143;
t1145 = t444.*t832;
t1146 = t806.*t813;
t1147 = t444.*t1047;
t1148 = t806.*t832;
t2025 = t444.*t831;
t2026 = t806.*t1048;
t1149 = t1119+t1147+t1148-t2025-t2026;
t1150 = (t197.*t593)./2.0;
t1151 = t8.*t729.*6.053757698066069e-1;
t1152 = t11.*t736.*1.18734317978;
t1153 = t13.*t736.*5.114817050334782e-3;
t1154 = t13.*t734.*1.18734317978;
t1240 = t2.*t727.*2.206;
t1241 = t11.*t734.*5.114817050334782e-3;
t1242 = t6.*t731.*6.053757698066069e-1;
t1155 = t187+t188+t189+t1151+t1152+t1153+t1154-t1240-t1241-t1242;
t1156 = t11.*t78.*5.114817050334782e-3;
t1157 = t11.*t84.*1.18734317978;
t1158 = t13.*t84.*5.114817050334782e-3;
t1295 = t13.*t78.*1.18734317978;
t1159 = t1156+t1157+t1158-t1295;
t1160 = (t148.*t1159)./2.0;
t1161 = t8.*t837.*1.139316919009596e-3;
t1162 = t11.*t880.*2.53401226709415e-4;
t1163 = t11.*t883.*8.169842925973351e-1;
t1164 = t3.*t727.*6.976304090397628e-20;
t1165 = t13.*t880.*8.169842925973351e-1;
t1545 = t13.*t883.*2.53401226709415e-4;
t1546 = t6.*t839.*1.139316919009596e-3;
t1166 = t531+t1161+t1162+t1163+t1164+t1165-t1545-t1546;
t1167 = t286.*t780;
t1168 = t425.*t788;
t1169 = t530.*t772;
t1170 = t8.*t837.*7.684130555159526e-1;
t1171 = t11.*t880.*8.979785040610579e-2;
t1172 = t11.*t883.*1.139316919009596e-3;
t1173 = t3.*t727.*4.705172944303244e-17;
t1174 = t13.*t880.*1.139316919009596e-3;
t1548 = t13.*t883.*8.979785040610579e-2;
t1549 = t6.*t839.*7.684130555159526e-1;
t1175 = t567+t1170+t1171+t1172+t1173+t1174-t1548-t1549;
t1176 = t8.*t837.*8.979785040610579e-2;
t1177 = t11.*t880.*4.876002456295764e-2;
t1178 = t11.*t883.*2.53401226709415e-4;
t1179 = t3.*t727.*5.498532503507515e-18;
t1180 = t13.*t880.*2.53401226709415e-4;
t1551 = t13.*t883.*4.876002456295764e-2;
t1552 = t6.*t839.*8.979785040610579e-2;
t1181 = t573+t1176+t1177+t1178+t1179+t1180-t1551-t1552;
t1182 = t124.*t1181;
t1547 = t164.*t1166;
t1550 = t101.*t1175;
t1183 = t1167+t1168+t1169+t1182-t1547-t1550;
t1184 = t57.*t640.*5.515;
t1185 = t586.*t727.*5.515;
t1401 = t20.*2.946606165491677e-33;
t1402 = t11.*t84.*1.917749226941314e-35;
t1186 = t584+t585+t587+t588+t589+t590+t591+t592+t1185-t1401-t1402;
t1189 = t3.*t727.*4.0e-1;
t1222 = t13.*t883.*2.152934142846781e-1;
t1239 = t8.*t837.*1.097689519141626e-1;
t1190 = t347+t964+t965+t966+t967+t1189-t1222-t1239;
t1191 = t164.*t673;
t1192 = t101.*t675;
t1193 = t129.*t425;
t1194 = t164.*t633;
t1195 = t100.*t286;
t1196 = t101.*t636;
t1197 = t134.*t530;
t1270 = t124.*t345;
t1198 = t1193+t1194+t1195+t1196+t1197-t1270;
t1199 = (t121.*t1198)./2.0;
t1200 = t11.*t78.*1.917749226941314e-35;
t1201 = t11.*t84.*4.451823873129729e-33;
t1202 = t13.*t84.*1.917749226941314e-35;
t1203 = t129.*t164;
t1204 = t101.*t134;
t1311 = t100.*t124;
t1205 = t1203+t1204-t1311;
t1206 = (t12.*t1205)./2.0;
t1207 = t8.*t62;
t1306 = t6.*t59;
t1208 = t58-t68+t1207-t1306;
t1209 = t6.*t59.*6.776895191416263e-2;
t1210 = t3.*t57.*4.149651502162508e-18;
t1309 = t2.*t21.*2.540928714850161e-34;
t1310 = t8.*t62.*6.776895191416263e-2;
t1211 = t289+t290+t291-t389+t1209+t1210-t1309-t1310;
t1212 = t11.*(t29+t30).*9.274373618014111e-4;
t1213 = t505+t506-t594-t643-t644+t645-t1187+t1212;
t1214 = t530.*t651.*5.515;
t1215 = t286.*t764;
t1416 = t164.*t667;
t1417 = t101.*t681;
t1216 = t661+t870+t871+t1215-t1416-t1417;
t1217 = t8.*t729.*2.269795582384779e-33;
t1218 = t11.*t736.*4.451823873129729e-33;
t1219 = t13.*t736.*1.917749226941314e-35;
t1220 = t13.*t734.*4.451823873129729e-33;
t1479 = t2.*t727.*8.271175201380145e-33;
t1480 = t11.*t734.*1.917749226941314e-35;
t1481 = t6.*t731.*2.269795582384779e-33;
t1221 = t693+t694+t695+t702+t1217+t1218+t1219+t1220-t1479-t1480-t1481;
t1224 = t3.*t727.*2.7582e-1;
t1357 = t8.*t837.*1.4967e-2;
t1225 = t244+t914+t915+t916+t1224-t1357;
t1226 = t8.*t729.*2.6117415e-2;
t1266 = t6.*t729.*2.799678e-4;
t1267 = t2.*t727.*4.813059e-1;
t1268 = t6.*t731.*2.6117415e-2;
t1269 = t8.*t731.*2.799678e-4;
t1227 = t165+t166+t167+t1226-t1266-t1267-t1268-t1269;
t1234 = (t197.*t292)./2.0;
t1247 = t6.*t837.*2.799678e-4;
t1248 = t3.*t727.*4.813059e-1;
t1249 = t6.*t839.*2.6117415e-2;
t1250 = t8.*t839.*2.799678e-4;
t1323 = t8.*t837.*2.6117415e-2;
t1251 = t328+t1247+t1248+t1249+t1250-t1323;
t1704 = t2.*t727.*1.20783555e-1;
t1705 = t3.*t727.*1.38974745e-2;
t1252 = t260+t261+t262-t1228-t1704-t1705;
t1253 = t3.*t727.*1.20783555e-1;
t1711 = t2.*t727.*1.38974745e-2;
t1254 = t219+t220+t1253-t1711;
t1255 = t2.*3.084900000000001e-3;
t1653 = t3.*2.6811e-2;
t1256 = t1255-t1653+3.468981871291444e-34;
t1257 = t2.*4.0e-1;
t1258 = t3.*2.449293598294706e-17;
t1259 = t505+t506+t507-t594-t845+t1212+t1257+t1258;
t1260 = t11.*t880.*1.18734317978;
t1261 = t11.*t883.*5.114817050334782e-3;
t1262 = t3.*t727.*2.206;
t1263 = t13.*t880.*5.114817050334782e-3;
t1264 = t6.*t839.*6.053757698066069e-1;
t1307 = t8.*t837.*6.053757698066069e-1;
t1308 = t13.*t883.*1.18734317978;
t1265 = t234+t1260+t1261+t1262+t1263+t1264-t1307-t1308;
t1271 = t2.*2.7582e-1;
t1272 = t3.*1.688910400704115e-17;
t1273 = t6.*(t3-t5).*1.6044e-4;
t1274 = t447+t448-t835+t1271+t1272+t1273;
t1275 = t2.*2.6811e-2;
t1276 = t3.*3.084900000000001e-3;
t1277 = t1275+t1276;
t1278 = t11.*t736.*5.114817050334782e-3;
t1279 = t11.*t734.*1.18734317978;
t1280 = t13.*t734.*5.114817050334782e-3;
t1981 = t13.*t736.*1.18734317978;
t1281 = t1278+t1279+t1280-t1981;
t1282 = t21.*5.342894225732869e-34;
t1283 = t20.*3.271579155863317e-50;
t1284 = t3.*t20.*9.18338008663387e-50;
t1285 = t8.*t729.*4.115676486645111e-34;
t1286 = t11.*t736.*8.072210105402954e-34;
t1287 = t13.*t736.*3.477333140419428e-36;
t1288 = t13.*t734.*8.072210105402954e-34;
t1289 = t57.*t586;
t1337 = t2.*t727.*1.499759782661858e-33;
t1338 = t11.*t734.*3.477333140419428e-36;
t1339 = t6.*t731.*4.115676486645111e-34;
t1290 = t1282+t1283+t1284+t1285+t1286+t1287+t1288+t1289-t1337-t1338-t1339;
t1291 = t6.*t839.*6.776895191416263e-2;
t1292 = t8.*t837;
t1294 = t6.*t839;
t1293 = t35+t838+t1292-t1294;
t1296 = t21.*3.271579155863317e-50;
t1297 = t3.*t21.*9.18338008663387e-50;
t1298 = t586.*t727;
t1299 = t11.*t78.*8.072210105402954e-34;
t1300 = t13.*t78.*3.477333140419428e-36;
t1301 = t6.*t65.*4.115676486645111e-34;
t1302 = t13.*(t79-t85).*8.072210105402954e-34;
t1303 = t8.*t67.*4.115676486645111e-34;
t1304 = t2.*t57.*1.499759782661858e-33;
t1353 = t20.*5.342894225732869e-34;
t1354 = t11.*t84.*3.477333140419428e-36;
t1305 = t1296+t1297+t1298+t1299+t1300+t1301+t1302+t1303+t1304-t1353-t1354;
t1312 = t11.*t883;
t1313 = t13.*t880;
t1314 = t1312+t1313;
t1315 = t129.*t1314;
t1316 = t633.*t766;
t1317 = t134.*t1293;
t1318 = t11.*t880;
t1392 = t13.*t883;
t1319 = t1318-t1392;
t1320 = t100.*t1319;
t1391 = t636.*t751;
t1393 = t345.*t762;
t1321 = t1315+t1316+t1317+t1320-t1391-t1393;
t1324 = t134.*t1208;
t1325 = t11.*t74;
t1395 = t13.*t72;
t1326 = t1325-t1395;
t1327 = t100.*t1326;
t1328 = t13.*t74;
t1329 = t11.*t72;
t1330 = t1328+t1329;
t1331 = t129.*t1330;
t1332 = t636.*t646;
t1333 = t13.*t757.*5.114817050334782e-3;
t1334 = t6.*t729.*6.053757698066069e-1;
t1335 = t8.*t731.*6.053757698066069e-1;
t1336 = t11.*t757.*1.18734317978;
t1340 = t6.*t729.*2.6117415e-2;
t1341 = t8.*t729.*2.799678e-4;
t1342 = t8.*t731.*2.6117415e-2;
t1787 = t6.*t731.*2.799678e-4;
t1343 = t1340+t1341+t1342-t1787;
t1344 = t21.*5.342894225732868e-34;
t1345 = t20.*3.271579155863317e-50;
t1346 = t57.*t859;
t1347 = t3.*t20.*6.332399738738385e-50;
t1348 = t8.*t729.*5.611726166775006e-35;
t1431 = t6.*t729.*6.015536488256711e-37;
t1432 = t2.*t727.*1.034159358134484e-33;
t1433 = t6.*t731.*5.611726166775006e-35;
t1434 = t8.*t731.*6.015536488256711e-37;
t1349 = t1344+t1345+t1346+t1347+t1348-t1431-t1432-t1433-t1434;
t1355 = t3.*t727.*2.6e-1;
t1356 = t445+t446+t447+t448-t835+t1273;
t1358 = t3.*t727.*1.3582e-1;
t1360 = t503+t504+t505+t506+t507-t594-t845+t1212;
t1362 = t21.*3.271579155863317e-50;
t1363 = t3.*t21.*6.332399738738385e-50;
t1364 = t6.*t65.*5.611726166775006e-35;
t1365 = t8.*t65.*6.015536488256711e-37;
t1366 = t727.*t859;
t1367 = t8.*t67.*5.611726166775006e-35;
t1368 = t2.*t57.*1.034159358134484e-33;
t1426 = t20.*5.342894225732868e-34;
t1427 = t6.*t67.*6.015536488256711e-37;
t1369 = t1362+t1363+t1364+t1365+t1366+t1367+t1368-t1426-t1427;
t1371 = t21.*8.725608443924892e-18;
t1419 = t20.*1.425e-1;
t1372 = t106+t107+t108+t109+t110-t283+t1371-t1419;
t1373 = t21.*1.425e-1;
t1374 = t20.*8.725608443924892e-18;
t1375 = t91+t840-t911-t912-t913-t979+t1373+t1374;
t1376 = t450.*t806;
t1377 = t121.*t978;
t1378 = t1376+t1377;
t1379 = t13.*t757.*1.917749226941314e-35;
t1380 = t6.*t729.*2.269795582384779e-33;
t1381 = t8.*t731.*2.269795582384779e-33;
t1382 = t11.*t757.*4.451823873129729e-33;
t1383 = t2.*t20.*9.18338008663387e-50;
t1384 = t11.*t880.*8.072210105402954e-34;
t1385 = t11.*t883.*3.477333140419428e-36;
t1386 = t3.*t727.*1.499759782661858e-33;
t1387 = t13.*t880.*3.477333140419428e-36;
t1388 = t6.*t839.*4.115676486645111e-34;
t1389 = t57.*t1259;
t1569 = t8.*t837.*4.115676486645111e-34;
t1570 = t13.*t883.*8.072210105402954e-34;
t1390 = t1383+t1384+t1385+t1386+t1387+t1388+t1389-t1569-t1570;
t1394 = (t57.*t1321)./2.0;
t1606 = t633.*t783;
t1607 = t345.*t775;
t1608 = t1324+t1327+t1331+t1332-t1606-t1607;
t1396 = (t727.*t1608)./2.0;
t1397 = t121.*t842;
t1398 = t67.*t429;
t1399 = t444.*t1360;
t1736 = t12.*t468;
t1400 = t1397+t1398+t1399-t1736;
t1403 = t450.*t806.*(3.49e2./2.0e2);
t1404 = t121.*t978.*(3.49e2./2.0e2);
t1405 = t1403+t1404;
t1406 = t2.*t20.*6.332399738738385e-50;
t1407 = t6.*t837.*6.015536488256711e-37;
t1408 = t3.*t727.*1.034159358134484e-33;
t1409 = t6.*t839.*5.611726166775006e-35;
t1410 = t8.*t839.*6.015536488256711e-37;
t1411 = t57.*t1274;
t1697 = t8.*t837.*5.611726166775006e-35;
t1412 = t1406+t1407+t1408+t1409+t1410+t1411-t1697;
t1413 = t429.*t444;
t1414 = t121.*t468;
t1415 = t1413+t1414;
t1418 = (t727.*t1216)./2.0;
t1420 = t57.*t1372.*(3.49e2./2.0e2);
t1692 = t727.*t1375.*(3.49e2./2.0e2);
t1421 = t1420-t1692;
t1422 = t836+t914+t915+t916-t1357+t1358;
t1423 = t57.*t1372;
t1689 = t727.*t1375;
t1424 = t1423-t1689;
t1428 = t962+t964+t965+t966+t967-t1222-t1239+t1355;
t1429 = t429.*t729.*5.515;
t1430 = t450.*t729.*(3.49e2./2.0e2);
t1435 = t21.*8.725608443924893e-18;
t1496 = t20.*1.425e-1;
t1436 = t141+t142+t143+t144+t145+t146+t147-t206+t1435-t1496;
t1437 = t21.*1.425e-1;
t1438 = t20.*8.725608443924893e-18;
t1439 = t156-t759+t807+t808+t809+t810-t830-t888+t1437+t1438;
t1440 = t462.*t727.*(3.49e2./2.0e2);
t1928 = t8.*t65.*9.792462161022385e-35;
t1441 = t906+t907+t908+t1440-t1928;
t1442 = t2.*t20.*9.157296440624334e-22;
t1443 = t8.*t837.*4.4101e-6;
t1444 = t3.*t727.*1.4955e-5;
t1752 = t6.*t837.*2.5506e-2;
t1753 = t6.*t839.*4.4101e-6;
t1754 = t8.*t839.*2.5506e-2;
t1445 = t1442+t1443+t1444-t1752-t1753-t1754;
t1446 = t15.*t1445;
t1447 = t12.*t1012;
t1448 = t6.*t837.*4.4101e-6;
t1449 = t3.*t727.*3.3204e-3;
t1450 = t6.*t839.*2.53e-2;
t1451 = t8.*t839.*4.4101e-6;
t1755 = t8.*t837.*2.53e-2;
t1452 = t898+t1448+t1449+t1450+t1451-t1755;
t1453 = t95.*t1452;
t1454 = t2.*t20.*2.092860147402869e-19;
t1455 = t3.*t727.*3.4179e-3;
t1456 = t6.*t839.*3.3204e-3;
t1756 = t6.*t837.*1.4955e-5;
t1757 = t8.*t837.*3.3204e-3;
t1758 = t8.*t839.*1.4955e-5;
t1457 = t1454+t1455+t1456-t1756-t1757-t1758;
t1750 = t31.*t1004;
t1751 = t243.*t1008;
t1759 = t121.*t1457;
t1458 = t1446+t1447+t1453-t1750-t1751-t1759;
t1459 = (t57.*t1458)./2.0;
t1460 = t520.*t727;
t1461 = t11.*t136.*8.072210105402954e-34;
t1462 = t13.*t136.*3.477333140419428e-36;
t1463 = t11.*t139.*3.477333140419428e-36;
t1464 = t6.*t67.*4.115676486645111e-34;
t1465 = t444.*t450;
t1466 = t121.*t527;
t1467 = t1465+t1466;
t1468 = t6.*t729.*9.792462161022385e-35;
t1469 = t8.*t729.*1.049711117200796e-36;
t1470 = t8.*t731.*9.792462161022385e-35;
t1931 = t6.*t731.*1.049711117200796e-36;
t1471 = t850+t1468+t1469+t1470-t1931;
t1472 = t429.*t806;
t1473 = t121.*t876;
t1474 = t1472+t1473;
t1475 = t121.*t1428;
t1476 = t429.*t729;
t1477 = t806.*t1360;
t1739 = t12.*t876;
t1478 = t1475+t1476+t1477-t1739;
t1482 = t2.*t21.*9.18338008663387e-50;
t1483 = t6.*t59.*4.115676486645111e-34;
t1484 = t13.*t74.*3.477333140419428e-36;
t1485 = t727.*t1259;
t1486 = t11.*t72.*3.477333140419428e-36;
t1487 = t11.*t74.*8.072210105402954e-34;
t1631 = t13.*t72.*8.072210105402954e-34;
t1632 = t8.*t62.*4.115676486645111e-34;
t1633 = t3.*t57.*1.499759782661858e-33;
t1488 = t1482+t1483+t1484+t1485+t1486+t1487-t1631-t1632-t1633;
t1489 = t462.*t727;
t1490 = t6.*t65.*6.015536488256711e-37;
t1491 = t6.*t67.*5.611726166775006e-35;
t1492 = t8.*t67.*6.015536488256711e-37;
t1785 = t8.*t65.*5.611726166775006e-35;
t1493 = t1489+t1490+t1491+t1492-t1785;
t1494 = t727.*t859.*(3.49e2./2.0e2);
t1558 = t20.*9.323350423903855e-34;
t1559 = t6.*t67.*1.049711117200796e-36;
t1495 = t855+t856+t857+t858+t860+t861+t1494-t1558-t1559;
t1497 = t57.*t1436.*5.515;
t1583 = t727.*t1439.*5.515;
t1498 = t1497-t1583;
t1499 = t57.*t1436;
t1588 = t727.*t1439;
t1500 = t1499-t1588;
t1501 = t520.*t727.*5.515;
t1502 = t2.*t21.*6.332399738738385e-50;
t1503 = t6.*t59.*5.611726166775006e-35;
t1504 = t8.*t59.*6.015536488256711e-37;
t1505 = t727.*t1274;
t1506 = t6.*t62.*6.015536488256711e-37;
t1663 = t8.*t62.*5.611726166775006e-35;
t1664 = t3.*t57.*1.034159358134484e-33;
t1507 = t1502+t1503+t1504+t1505+t1506-t1663-t1664;
t1508 = t13.*t757.*3.477333140419428e-36;
t1509 = t6.*t729.*4.115676486645111e-34;
t1510 = t13.*(t750-t754).*8.072210105402954e-34;
t1511 = t57.*t520;
t1512 = t8.*t731.*4.115676486645111e-34;
t1513 = t11.*t757.*8.072210105402954e-34;
t1797 = t11.*t758.*3.477333140419428e-36;
t1514 = t1508+t1509+t1510+t1511+t1512+t1513-t1797;
t1515 = t6.*t729.*5.611726166775006e-35;
t1516 = t8.*t729.*6.015536488256711e-37;
t1517 = t57.*t462;
t1518 = t8.*t731.*5.611726166775006e-35;
t1793 = t6.*t731.*6.015536488256711e-37;
t1519 = t1515+t1516+t1517+t1518-t1793;
t1520 = t8.*t729.*9.792462161022385e-35;
t1565 = t6.*t729.*1.049711117200796e-36;
t1566 = t2.*t727.*1.804608079944675e-33;
t1567 = t6.*t731.*9.792462161022385e-35;
t1568 = t8.*t731.*1.049711117200796e-36;
t1521 = t917+t918+t920+t921+t1520-t1565-t1566-t1567-t1568;
t1531 = (t727.*t961)./2.0;
t1532 = t1292-t1294;
t1533 = t379.*t806;
t1534 = t120.*t883;
t1535 = t321.*t734;
t1536 = t309.*t729;
t2076 = t242.*t1532;
t2077 = t366.*t758;
t1537 = t1533+t1534+t1535+t1536-t2076-t2077;
t1538 = t1207-t1306;
t1539 = t139.*t366;
t1540 = t72.*t120;
t1541 = t67.*t309;
t1542 = t379.*t444;
t1543 = t84.*t321;
t2078 = t242.*t1538;
t1544 = t1539+t1540+t1541+t1542+t1543-t2078;
t1553 = (t57.*t1183)./2.0;
t1554 = t444.*t1356;
t1555 = t67.*t450;
t1556 = t121.*t902;
t1747 = t12.*t527;
t1557 = t1554+t1555+t1556-t1747;
t1561 = t806.*t1356;
t1562 = t450.*t729;
t1563 = t121.*t1422;
t1743 = t12.*t978;
t1564 = t1561+t1562+t1563-t1743;
t1571 = t751.*t1213;
t1584 = t2.*t20.*2.540928714850161e-34;
t1585 = t8.*t837.*6.776895191416263e-2;
t1586 = t3.*t727.*4.149651502162508e-18;
t1587 = t964+t965+t966-t1222+t1291-t1584-t1585-t1586;
t1572 = t101.*t1587;
t1573 = t530.*t834;
t1574 = t603.*t1293;
t1575 = t1571+t1572+t1573+t1574;
t1576 = t640.*t727;
t1577 = t11.*t78.*3.477333140419428e-36;
t1578 = t11.*t84.*8.072210105402954e-34;
t1579 = t13.*t84.*3.477333140419428e-36;
t1800 = t13.*t78.*8.072210105402954e-34;
t1580 = t1576+t1577+t1578+t1579-t1800;
t1581 = (t806.*t1183)./2.0;
t1582 = (t806.*t1321)./2.0;
t1589 = t101.*t651;
t1807 = t603.*t646;
t1590 = t1589-t1807;
t1591 = t2.*t21.*5.06463411777858e-49;
t1592 = t6.*t59.*2.269795582384779e-33;
t1593 = t13.*t74.*1.917749226941314e-35;
t1594 = t727.*t1259.*5.515;
t1595 = t11.*t72.*1.917749226941314e-35;
t1596 = t11.*t74.*4.451823873129729e-33;
t1649 = t13.*t72.*4.451823873129729e-33;
t1650 = t8.*t62.*2.269795582384779e-33;
t1651 = t3.*t57.*8.271175201380145e-33;
t1597 = t1591+t1592+t1593+t1594+t1595+t1596-t1649-t1650-t1651;
t1598 = t11.*t736.*3.477333140419428e-36;
t1599 = t11.*t734.*8.072210105402954e-34;
t1600 = t13.*t734.*3.477333140419428e-36;
t1601 = t57.*t640;
t1801 = t13.*t736.*8.072210105402954e-34;
t1602 = t1598+t1599+t1600+t1601-t1801;
t1809 = t124.*t764;
t1603 = t1191+t1192-t1809;
t1604 = t640.*t727.*5.515;
t2011 = t13.*t78.*4.451823873129729e-33;
t1605 = t1200+t1201+t1202+t1604-t2011;
t1609 = t646.*t1213.*5.515;
t1971 = t603.*t1208.*5.515;
t1972 = t101.*t1211.*5.515;
t1610 = t1214+t1609-t1971-t1972;
t1611 = t101.*t834;
t1612 = t2.*t20.*5.06463411777858e-49;
t1613 = t11.*t880.*4.451823873129729e-33;
t1614 = t11.*t883.*1.917749226941314e-35;
t1615 = t3.*t727.*8.271175201380145e-33;
t1616 = t13.*t880.*1.917749226941314e-35;
t1617 = t6.*t839.*2.269795582384779e-33;
t1618 = t57.*t1259.*5.515;
t1695 = t8.*t837.*2.269795582384779e-33;
t1696 = t13.*t883.*4.451823873129729e-33;
t1619 = t1612+t1613+t1614+t1615+t1616+t1617+t1618-t1695-t1696;
t1620 = t57.*t292.*5.515;
t1699 = t727.*t1190.*5.515;
t1621 = t1620-t1699;
t1622 = t57.*t292;
t1698 = t727.*t1190;
t1623 = t1622-t1698;
t1624 = (t67.*t1118)./2.0;
t1625 = (t729.*t1076)./2.0;
t1626 = t11.*t736.*1.917749226941314e-35;
t1627 = t11.*t734.*4.451823873129729e-33;
t1628 = t13.*t734.*1.917749226941314e-35;
t2018 = t13.*t736.*4.451823873129729e-33;
t1629 = t1184+t1626+t1627+t1628-t2018;
t1630 = (t444.*t1216)./2.0;
t1634 = t751.*t1213.*5.515;
t1635 = t530.*t834.*5.515;
t1636 = t603.*t1293.*5.515;
t1637 = t101.*t772;
t1638 = t164.*t788;
t1808 = t124.*t780;
t1639 = t1637+t1638-t1808;
t1640 = t646.*t1213;
t1641 = t530.*t651;
t1642 = t2.*t20.*1.105003754409848e-49;
t1643 = t6.*t837.*1.049711117200796e-36;
t1644 = t3.*t727.*1.804608079944675e-33;
t1645 = t6.*t839.*9.792462161022385e-35;
t1646 = t8.*t839.*1.049711117200796e-36;
t1647 = t57.*t1274.*(3.49e2./2.0e2);
t1720 = t8.*t837.*9.792462161022385e-35;
t1648 = t1642+t1643+t1644+t1645+t1646+t1647-t1720;
t1652 = t2.*t20.*7.082452307314206e-52;
t1654 = t57.*t1256;
t1655 = t2.*t727.*1.005251488323677e-34;
t1656 = t3.*t727.*1.156652238383391e-35;
t1712 = t21.*3.468981871291444e-34;
t1713 = t20.*2.124138772488631e-50;
t1714 = t3.*t20.*6.155390087568518e-51;
t1657 = t1652+t1654+t1655+t1656-t1712-t1713-t1714;
t1658 = t21.*2.124138772488631e-50;
t1659 = t3.*t21.*6.155390087568518e-51;
t1660 = t2.*t57.*1.005251488323677e-34;
t1661 = t3.*t57.*1.156652238383391e-35;
t1700 = t20.*3.468981871291444e-34;
t1701 = t2.*t21.*7.082452307314206e-52;
t1702 = t727.*t1256;
t1662 = t1658+t1659+t1660+t1661-t1700-t1701-t1702;
t1665 = t3.*t727.*2.6811e-2;
t1667 = t2.*t727.*3.0849e-3;
t1666 = t256+t257+t1665-t1667;
t1668 = t21.*5.665277325195614e-18;
t1669 = t20.*(-9.252100000000001e-2)+t272+t273+t274-t1231+t1668;
t1670 = t21.*9.252100000000001e-2;
t1671 = t20.*5.665277325195614e-18;
t1728 = t2.*t727.*2.6811e-2;
t1729 = t3.*t727.*3.0849e-3;
t1672 = t223-t1223+t1670+t1671-t1728-t1729;
t1673 = t2.*t20.*6.155390087568518e-51;
t1674 = t3.*t20.*7.082452307314206e-52;
t1675 = t3.*t727.*1.005251488323677e-34;
t1676 = t57.*t1277;
t1703 = t2.*t727.*1.156652238383391e-35;
t1677 = t1673+t1674+t1675+t1676-t1703;
t1678 = t2.*t21.*6.155390087568518e-51;
t1679 = t3.*t21.*7.082452307314206e-52;
t1680 = t2.*t57.*1.156652238383391e-35;
t1681 = t727.*t1277;
t1730 = t3.*t57.*1.005251488323677e-34;
t1682 = t1678+t1679+t1680+t1681-t1730;
t1683 = t2.*t21.*1.105003754409848e-49;
t1684 = t6.*t59.*9.792462161022385e-35;
t1685 = t8.*t59.*1.049711117200796e-36;
t1686 = t727.*t1274.*(3.49e2./2.0e2);
t1687 = t6.*t62.*1.049711117200796e-36;
t1721 = t8.*t62.*9.792462161022385e-35;
t1722 = t3.*t57.*1.804608079944675e-33;
t1688 = t1683+t1684+t1685+t1686+t1687-t1721-t1722;
t1690 = t57.*t372.*(3.49e2./2.0e2);
t1691 = t1690-t727.*t1225.*(3.49e2./2.0e2);
t1693 = t57.*t372;
t1940 = t727.*t1225;
t1694 = t1693-t1940;
t1706 = t2.*t20.*3.19064476444505e-51;
t1707 = t57.*t1256.*(9.01e2./2.0e2);
t1708 = t2.*t727.*4.528657954898164e-34;
t1709 = t3.*t727.*5.210718333917177e-35;
t1710 = t20.*(-9.569245170061283e-50)-t21.*1.562776333016795e-33+t1706+t1707+t1708+t1709-t3.*t20.*2.773003234449617e-50;
t1715 = t2.*t21.*2.773003234449617e-50;
t1716 = t3.*t21.*3.19064476444505e-51;
t1717 = t2.*t57.*5.210718333917177e-35;
t1718 = t727.*t1277.*(9.01e2./2.0e2);
t1719 = t1715+t1716+t1717+t1718-t3.*t57.*4.528657954898164e-34;
t1723 = t2.*t20.*2.773003234449617e-50;
t1724 = t3.*t20.*3.19064476444505e-51;
t1725 = t3.*t727.*4.528657954898164e-34;
t1726 = t57.*t1277.*(9.01e2./2.0e2);
t1727 = t1723+t1724+t1725+t1726-t2.*t727.*5.210718333917177e-35;
t1731 = t21.*9.569245170061283e-50;
t1732 = t3.*t21.*2.773003234449617e-50;
t1733 = t2.*t57.*4.528657954898164e-34;
t1734 = t3.*t57.*5.210718333917177e-35;
t1735 = t20.*(-1.562776333016795e-33)+t1731+t1732+t1733+t1734-t2.*t21.*3.19064476444505e-51-t727.*t1256.*(9.01e2./2.0e2);
t1737 = t444.*t1360.*5.515;
t1738 = t843+t844-t1560+t1737;
t1740 = t121.*t1428.*5.515;
t1741 = t806.*t1360.*5.515;
t1795 = t12.*t876.*5.515;
t1742 = t1429+t1740+t1741-t1795;
t1744 = t806.*t1356.*(3.49e2./2.0e2);
t1745 = t121.*t1422.*(3.49e2./2.0e2);
t1780 = t12.*t978.*(3.49e2./2.0e2);
t1746 = t1430+t1744+t1745-t1780;
t1748 = t444.*t1356.*(3.49e2./2.0e2);
t1749 = t899+t903-t1425+t1748;
t1760 = t527.*t806.*(3.49e2./2.0e2);
t1761 = t67.*t978;
t1762 = t444.*t1422;
t1939 = t444.*t978.*(3.49e2./2.0e2);
t1763 = t1760-t1939;
t2138 = t806.*t902;
t2139 = t527.*t729;
t1764 = t1761+t1762-t2138-t2139;
t1765 = t527.*t806;
t1766 = t67.*t978.*(3.49e2./2.0e2);
t1767 = t444.*t1422.*(3.49e2./2.0e2);
t2111 = t444.*t978;
t1768 = t1765-t2111;
t1924 = t806.*t902.*(3.49e2./2.0e2);
t1925 = t527.*t729.*(3.49e2./2.0e2);
t1769 = t1766+t1767-t1924-t1925;
t1770 = t468.*t806.*5.515;
t1866 = t444.*t876.*5.515;
t1771 = t1770-t1866;
t1772 = t67.*t876;
t1773 = t444.*t1428;
t1960 = t468.*t729;
t1961 = t806.*t842;
t1774 = t1772+t1773-t1960-t1961;
t1775 = t468.*t806;
t1962 = t444.*t876;
t1776 = t1775-t1962;
t1777 = t67.*t876.*5.515;
t1778 = t444.*t1428.*5.515;
t1856 = t468.*t729.*5.515;
t1857 = t806.*t842.*5.515;
t1779 = t1777+t1778-t1856-t1857;
t1781 = t13.*(t750-t754).*1.18734317978;
t2021 = t11.*t758.*5.114817050334782e-3;
t1782 = t1333+t1334+t1335+t1336+t1781-t2021;
t1783 = (t1290.*t1782)./2.0;
t1872 = t8.*t65.*4.115676486645111e-34;
t1873 = t13.*t139.*8.072210105402954e-34;
t1909 = t1460+t1461+t1462+t1463+t1464-t1872-t1873;
t1784 = (t197.*t1909)./2.0;
t1786 = (t177.*t1493)./2.0;
t1788 = (t1343.*t1349)./2.0;
t1789 = (t1305.*(t985+t986+t987+t988-t1351-t1352))./2.0;
t1790 = t12.*t309.*1.874699728327322e-33;
t1791 = t15.*t321.*1.874699728327322e-33;
t1792 = t124.*t345.*1.874699728327322e-33;
t1794 = (t1227.*t1519)./2.0;
t1796 = t95.*t366.*1.874699728327322e-33;
t1798 = (t1155.*t1514)./2.0;
t1799 = (t983.*t1369)./2.0;
t1802 = t13.*(t750-t754).*2.152934142846781e-1;
t1803 = t825+t826+t922+t923-t995+t1802;
t1804 = t57.*t829;
t1805 = t651.*t751.*5.515;
t1944 = t646.*t834.*5.515;
t1806 = t1805-t1944;
t1810 = t11.*t736.*1.139316919009596e-3;
t1811 = t11.*t734.*8.979785040610579e-2;
t1812 = t13.*t734.*1.139316919009596e-3;
t1945 = t13.*t736.*8.979785040610579e-2;
t1813 = t1810+t1811+t1812-t1945;
t1814 = t11.*t736.*8.169842925973351e-1;
t1815 = t13.*t734.*8.169842925973351e-1;
t1816 = -t777+t796+t1814+t1815;
t1817 = t164.*t780;
t1818 = t124.*t788;
t1819 = t11.*t734.*4.876002456295764e-2;
t1948 = t13.*t736.*4.876002456295764e-2;
t1820 = t784+t786+t1819-t1948;
t1821 = t124.*t1820;
t1946 = t101.*t1813;
t1947 = t164.*t1816;
t1822 = t1817+t1818+t1821-t1946-t1947;
t1823 = (t57.*t1822)./2.0;
t1825 = t164.*t764;
t1949 = t101.*t1067;
t1950 = t164.*t1070;
t1827 = t1071+t1073+t1825-t1949-t1950;
t1828 = (t727.*t1827)./2.0;
t1832 = t134.*t1208.*3.749399456654644e-33;
t1833 = t788.*t1330;
t1834 = t775.*t1181;
t1835 = t783.*t1166;
t1836 = t772.*t1208;
t1837 = t780.*t1326;
t1970 = t646.*t1175;
t1838 = t1833+t1834+t1835+t1836+t1837-t1970;
t1839 = t57.*t1838;
t1840 = t100.*t1326.*3.749399456654644e-33;
t1841 = t667.*t783;
t1842 = t675.*t1208;
t1843 = t673.*t1330;
t1844 = t660.*t775;
t1845 = t764.*t1326;
t1969 = t646.*t681;
t1846 = t1841+t1842+t1843+t1844+t1845-t1969;
t1847 = t727.*t1846;
t1848 = t129.*t1330.*3.749399456654644e-33;
t1849 = t636.*t646.*3.749399456654644e-33;
t2146 = t633.*t783.*3.749399456654644e-33;
t2147 = t345.*t775.*3.749399456654644e-33;
t1850 = t1832+t1839+t1840+t1847+t1848+t1849-t2146-t2147;
t1853 = t825+t826-t995+t1122+t1123+t1802;
t1854 = t651.*t751;
t1987 = t646.*t834;
t1855 = t1854-t1987;
t1867 = t834.*t1208;
t1868 = t751.*t1211;
t1869 = t651.*t1293;
t1870 = t646.*t1587;
t1871 = t1867+t1868+t1869+t1870;
t1874 = t57.*t593;
t1968 = t727.*t805;
t1875 = t1874-t1968;
t1876 = t660.*t762;
t1877 = t681.*t751;
t1878 = t675.*t1293;
t1879 = t764.*t1319;
t1880 = t673.*t1314;
t1951 = t667.*t766;
t1881 = t1876+t1877+t1878+t1879+t1880-t1951;
t1882 = t727.*t1881;
t1883 = t129.*t1314.*3.749399456654644e-33;
t1884 = t633.*t766.*3.749399456654644e-33;
t1885 = t134.*t1293.*3.749399456654644e-33;
t1886 = t751.*t1175;
t1887 = t772.*t1293;
t1888 = t780.*t1319;
t1889 = t788.*t1314;
t1890 = t762.*t1181;
t1952 = t766.*t1166;
t1891 = t1886+t1887+t1888+t1889+t1890-t1952;
t1892 = t57.*t1891;
t1893 = t100.*t1319.*3.749399456654644e-33;
t2115 = t636.*t751.*3.749399456654644e-33;
t2116 = t345.*t762.*3.749399456654644e-33;
t1894 = t1882+t1883+t1884+t1885+t1892+t1893-t2115-t2116;
t1895 = t57.*t1047;
t1896 = t727.*t1048;
t2044 = t129.*t766.*3.749399456654644e-33;
t1897 = t1030+t1031+t1895+t1896-t2044;
t1976 = t13.*t757.*2.53401226709415e-4;
t1977 = t13.*(t750-t754).*4.876002456295764e-2;
t1978 = t11.*t757.*4.876002456295764e-2;
t2208 = t1129+t1130+t1131-t1976-t1977-t1978;
t1903 = t124.*t2208;
t1975 = t101.*t1127;
t1979 = t164.*t1136;
t1980 = t456.*t788;
t1907 = t1128+t1132+t1903-t1975-t1979-t1980;
t1908 = (t806.*t1907)./2.0;
t2005 = t603.*t1208;
t2006 = t101.*t1211;
t1910 = t1640+t1641-t2005-t2006;
t2004 = t603.*t751;
t1911 = t1611-t2004;
t1912 = t57.*t416;
t2081 = t727.*t993;
t1913 = t1912-t2081;
t1914 = (t1421.*t1913)./2.0;
t1915 = t57.*t416.*(3.49e2./2.0e2);
t2082 = t727.*t993.*(3.49e2./2.0e2);
t1916 = t1915-t2082;
t1917 = (t1424.*t1916)./2.0;
t1918 = t13.*(t750-t754).*4.451823873129729e-33;
t2083 = t11.*t758.*1.917749226941314e-35;
t1919 = t887+t1379+t1380+t1381+t1382+t1918-t2083;
t1920 = (t1290.*t1919)./2.0;
t1921 = t129.*t425.*3.749399456654644e-33;
t1922 = t164.*t633.*3.749399456654644e-33;
t1923 = t727.*t1216;
t1926 = t57.*t829.*5.515;
t2084 = t727.*t1803.*5.515;
t2166 = t1926-t2084;
t1927 = (t1500.*t2166)./2.0;
t1929 = (t1369.*t1441)./2.0;
t1930 = t100.*t286.*3.749399456654644e-33;
t1932 = (t1349.*t1471)./2.0;
t1933 = t101.*t636.*3.749399456654644e-33;
t1934 = t134.*t530.*3.749399456654644e-33;
t1935 = (t1493.*t1495)./2.0;
t2085 = t8.*t65.*2.269795582384779e-33;
t2086 = t13.*t139.*4.451823873129729e-33;
t2165 = t969+t970+t971+t972+t1501-t2085-t2086;
t1936 = (t1305.*t2165)./2.0;
t1937 = (t1221.*t1514)./2.0;
t1938 = (t1519.*t1521)./2.0;
t1941 = t57.*t1183;
t1943 = t727.*t1803;
t1942 = t1804-t1943;
t1953 = t444.*t805.*5.515;
t1954 = t1953-t593.*t806.*5.515;
t1955 = (t1500.*t1954)./2.0;
t2310 = t751.*t823.*5.515;
t2311 = t101.*t1853.*5.515;
t1956 = t1120+t1121-t2310-t2311;
t1957 = t651.*t734.*5.515;
t1958 = t84.*t834.*5.515;
t2341 = t751.*t1852.*5.515;
t2342 = t646.*t1853.*5.515;
t1959 = t1957+t1958-t2341-t2342;
t1963 = t834.*t1208.*5.515;
t1964 = t751.*t1211.*5.515;
t1965 = (t49-t63-t64+t137+t138-t642).*(t964+t965+t966-t1222+t1291-t1584-t1585-t1586).*5.515;
t1966 = t651.*t1293.*5.515;
t1967 = t1963+t1964+t1965+t1966;
t1973 = t101.*(t964+t965+t966-t1222+t1291-t1584-t1585-t1586).*5.515;
t1974 = t1634+t1635+t1636+t1973;
t1982 = (t1281.*t1290)./2.0;
t1983 = (t1110.*t1190)./2.0;
t1984 = (t1155.*t1602)./2.0;
t1985 = (t148.*t1610)./2.0;
t1986 = (t197.*t1580)./2.0;
t1988 = t729.*t814;
t1989 = t764.*(t1325-t1395);
t1990 = t1841+t1842+t1843+t1844-t1969+t1989;
t1991 = t444.*t1990;
t1992 = t780.*(t1325-t1395);
t1993 = t1833+t1834+t1835+t1836-t1970+t1992;
t1994 = t806.*t1993;
t1995 = t67.*t813;
t1996 = t121.*(t1324+t1327+t1331+t1332-t1606-t1607);
t2189 = t12.*t1118;
t1997 = t1988+t1991+t1994+t1995+t1996-t2189;
t1998 = t121.*t1321;
t1999 = t67.*t1048;
t2000 = t444.*t1881;
t2001 = t729.*t1047;
t2002 = t806.*t1891;
t2171 = t12.*t1076;
t2003 = t1998+t1999+t2000+t2001+t2002-t2171;
t2007 = (t1186.*t1580)./2.0;
t2008 = t806.*t1183;
t2009 = (t1221.*t1602)./2.0;
t2010 = t121.*t1198;
t2012 = (t1305.*t1605)./2.0;
t2013 = (t1498.*t1875)./2.0;
t2014 = t57.*t593.*5.515;
t2188 = t727.*t805.*5.515;
t2015 = t2014-t2188;
t2016 = (t1500.*t2015)./2.0;
t2017 = t12.*t1205;
t2019 = (t1290.*t1629)./2.0;
t2020 = t444.*t1216;
t2022 = (t727.*t1144)./2.0;
t2023 = t806.*(t801-t811-t812+t815+t816-t1032);
t2024 = t1077+t1145+t1146+t2023-t444.*t814;
t2027 = (t57.*t1149)./2.0;
t2029 = (t851.*t1343)./2.0;
t2030 = (t993.*t1227)./2.0;
t2031 = t1026+t1027+t1043-t1049-t1050+t1054;
t2032 = t1023+t1024+t1025+t1041+t1042-t1053;
t2033 = t57.*t1045;
t2034 = t11.*t758;
t2097 = t13.*t757;
t2209 = t2034-t2097;
t2035 = t129.*t2209;
t2036 = t13.*t758;
t2037 = t11.*t757;
t2038 = t2036+t2037;
t2039 = t442.*t762;
t2040 = t398.*t751;
t2041 = t134.*t734;
t2098 = t100.*t2038;
t2099 = t488.*t766;
t2042 = t2035+t2039+t2040+t2041-t2098-t2099;
t2043 = t57.*(t801-t811-t812+t815+t816-t1032);
t2045 = t727.*t1047;
t2046 = t818+t820+t1037-t1038+t2045-t57.*t1048-t727.*t831;
t2047 = (t57.*t2046)./2.0;
t2048 = t13.*t136;
t2049 = t11.*t139;
t2050 = t2048+t2049;
t2051 = t442.*t775;
t2052 = t488.*t783;
t2053 = t11.*t136;
t2122 = t13.*t139;
t2054 = t2053-t2122;
t2055 = t84.*t134;
t2120 = t129.*t2050;
t2121 = t398.*t646;
t2123 = t100.*t2054;
t2056 = t2051+t2052+t2055-t2120-t2121-t2123;
t2057 = t727.*t1052;
t2058 = t57.*t1051;
t2238 = t309.*t806.*3.749399456654644e-33;
t2059 = t1039+t1040+t2057+t2058-t2238;
t2060 = (t727.*t2059)./2.0;
t2061 = t727.*t1045;
t2062 = t57.*t1046;
t2063 = (t727.*t1897)./2.0;
t2064 = t727.*t1051;
t2065 = t57.*t2032;
t2066 = t727.*t2031;
t2281 = t309.*t444.*3.749399456654644e-33;
t2282 = t139.*t242.*3.749399456654644e-33;
t2293 = t57.*t1052;
t2067 = t1055+t2064+t2065+t2066-t2281-t2282-t2293;
t2068 = (t57.*t2067)./2.0;
t2069 = (t1251.*t1378)./2.0;
t2070 = t120.*(t29+t30).*1.874699728327322e-33;
t2071 = (t281.*t1467)./2.0;
t2072 = (t177.*t1557)./2.0;
t2073 = (t1265.*t1474)./2.0;
t2074 = (t1155.*t1478)./2.0;
t2075 = (t359.*t1415)./2.0;
t2079 = (t1227.*t1564)./2.0;
t2080 = (t197.*t1400)./2.0;
t2087 = t129.*t425.*7.02899814278107e-66;
t2088 = t100.*t392.*3.749399456654644e-33;
t2089 = t121.*t993;
t2090 = t462.*t806;
t2091 = t2089+t2090;
t2092 = t121.*t416;
t2093 = t444.*t462;
t2094 = t2092+t2093;
t2095 = t15.*t242.*3.749399456654644e-33;
t2096 = t164.*t633.*7.02899814278107e-66;
t2100 = t95.*t120.*3.749399456654644e-33;
t2101 = t444.*t520;
t2102 = t121.*(t403+t404+t405+t406-t833-t853);
t2103 = t2101+t2102;
t2104 = t121.*t1803;
t2105 = t520.*t806;
t2106 = t2104+t2105;
t2107 = t120.*t139;
t2108 = t139.*t421;
t2109 = t84.*t242;
t2260 = t436.*t444;
t2110 = t2107+t2108+t2109-t2260-t84.*t388;
t2112 = t95.*t421.*3.749399456654644e-33;
t2113 = t727.*t1216.*1.874699728327322e-33;
t2114 = t121.*t436.*3.749399456654644e-33;
t2117 = t124.*t442.*3.749399456654644e-33;
t2118 = t100.*t286.*7.02899814278107e-66;
t2119 = t57.*t1458.*1.874699728327322e-33;
t2124 = t379.*t806.*3.749399456654644e-33;
t2125 = t120.*t883.*3.749399456654644e-33;
t2126 = t734.*t1445;
t2127 = t729.*t1012;
t2128 = t806.*t1457;
t2377 = t1008.*t1532;
t2378 = t758.*t1452;
t2379 = t883.*t1004;
t2129 = t2126+t2127+t2128-t2377-t2378-t2379;
t2130 = t734.*t935;
t2131 = t806.*t954;
t2132 = t883.*t960;
t2133 = t930.*t1532;
t2134 = t321.*t734.*3.749399456654644e-33;
t2135 = t309.*t729.*3.749399456654644e-33;
t2136 = t101.*t636.*7.02899814278107e-66;
t2137 = t15.*t134.*3.749399456654644e-33;
t2140 = t134.*t530.*7.02899814278107e-66;
t2141 = t388.*t734;
t2142 = t120.*t758;
t2143 = t421.*t758;
t2144 = t436.*t806;
t2291 = t242.*t734;
t2292 = t2141+t2142+t2143+t2144-t2291;
t2145 = t57.*t2292;
t2148 = t727.*t961.*1.874699728327322e-33;
t2149 = t121.*t379.*7.02899814278107e-66;
t2150 = t930.*t1538;
t2151 = t444.*t954;
t2152 = t84.*t935;
t2153 = t72.*t960;
t2397 = t67.*t942;
t2398 = t139.*t948;
t2154 = t727.*(t2150+t2151+t2152+t2153-t2397-t2398);
t2155 = t139.*t366.*3.749399456654644e-33;
t2156 = t72.*t120.*3.749399456654644e-33;
t2157 = t67.*t309.*3.749399456654644e-33;
t2158 = t379.*t444.*3.749399456654644e-33;
t2159 = t67.*t1012;
t2160 = t444.*t1457;
t2161 = t139.*t1452;
t2162 = t84.*t1445;
t2399 = t72.*t1004;
t2400 = t1008.*t1538;
t2163 = t2159+t2160+t2161+t2162-t2399-t2400;
t2164 = t57.*t1183.*1.874699728327322e-33;
t2167 = (t714.*t1400)./2.0;
t2168 = t15.*t651;
t2169 = t101.*t1852;
t2300 = t646.*t823;
t2170 = t2168+t2169-t2300-t84.*t603;
t2172 = (t57.*t2003)./2.0;
t2173 = t121.*t593;
t2174 = t444.*t640;
t2175 = t2173+t2174;
t2176 = t67.*t1603.*1.874699728327322e-33;
t2177 = (t806.*t2042)./2.0;
t2178 = t121.*t805;
t2179 = t640.*t806;
t2180 = t2178+t2179;
t2181 = (t1776.*t1967)./2.0;
t2182 = t100.*t766;
t2183 = t613.*t766;
t2184 = t129.*t762;
t2437 = t653.*t762;
t2438 = t598.*t751;
t2185 = t2182+t2183+t2184-t2437-t2438;
t2186 = t603.*t734;
t2187 = t15.*t834;
t2190 = (t727.*t1997)./2.0;
t2191 = (t1474.*t1974)./2.0;
t2192 = t729.*t1639.*1.874699728327322e-33;
t2193 = t613.*t783;
t2194 = t653.*t775;
t2195 = t100.*t783;
t2444 = t598.*t646;
t2196 = t2193+t2194+t2195-t2444-t129.*t775;
t2197 = (t727.*t2196)./2.0;
t2198 = (t444.*t2056)./2.0;
t2308 = t751.*t823;
t2309 = t101.*t1853;
t2199 = t2186+t2187-t2308-t2309;
t2200 = (t851.*t1471)./2.0;
t2201 = (t416.*t1495)./2.0;
t2202 = (t111.*t1441)./2.0;
t2203 = (t993.*t1521)./2.0;
t2204 = t416.*t806;
t2393 = t444.*t993;
t2205 = t2204-t2393;
t2206 = t806.*t829;
t2211 = t6.*t67.*2.53e-2;
t2229 = t8.*t65.*2.53e-2;
t2212 = t998+t1000+t2211-t2229;
t2213 = t6.*t65.*1.4955e-5;
t2214 = t8.*t65.*3.3204e-3;
t2215 = t8.*t67.*1.4955e-5;
t2230 = t6.*t67.*3.3204e-3;
t2216 = t2213+t2214+t2215-t2230;
t2217 = t6.*t65.*2.5506e-2;
t2218 = t8.*t67.*2.5506e-2;
t2219 = -t927+t1006+t2217+t2218;
t2220 = t6.*t729.*2.53e-2;
t2221 = t8.*t731.*2.53e-2;
t2222 = -t1002+t1017+t2220+t2221;
t2223 = t6.*t729.*3.3204e-3;
t2224 = t6.*t731.*1.4955e-5;
t2225 = t8.*t731.*3.3204e-3;
t2232 = t8.*t729.*1.4955e-5;
t2226 = t2223+t2224+t2225-t2232;
t2227 = t8.*t729.*2.5506e-2;
t2231 = t6.*t731.*2.5506e-2;
t2228 = t1019+t1022+t2227-t2231;
t2233 = -t79+t85;
t2234 = t11.*t2233.*2.53401226709415e-4;
t2246 = t13.*t2233.*4.876002456295764e-2;
t2235 = t614+t615+t616+t617+t618-t668-t669-t671+t2234-t2246;
t2236 = t11.*t2233.*1.139316919009596e-3;
t2249 = t13.*t2233.*8.979785040610579e-2;
t2237 = t626+t627+t628+t629+t630-t737-t738-t740+t2236-t2249;
t2239 = t444.*t520.*5.515;
t2240 = t121.*(t403+t404+t405+t406-t833-t853).*5.515;
t2241 = t2239+t2240;
t2242 = t11.*t2233.*9.274373618014111e-4;
t2243 = t121.*t993.*(3.49e2./2.0e2);
t2244 = t462.*t806.*(3.49e2./2.0e2);
t2245 = t2243+t2244;
t2247 = t11.*t2233.*8.169842925973351e-1;
t2256 = t13.*t2233.*2.53401226709415e-4;
t2248 = t621+t622+t623+t624+t625-t715-t716-t718+t2247-t2256;
t2253 = t13.*t2233;
t2250 = t773-t2253;
t2251 = t11.*t2233;
t2252 = t782+t2251;
t2254 = t780.*t2250;
t2255 = t788.*t2252;
t2257 = t646.*t2237;
t2258 = t2235.*t2250;
t2259 = t2248.*t2252;
t2261 = -t2257+t2258+t2259;
t2262 = -t819+t2254+t2255;
t2263 = t815+t816-t1032+t2257-t2258-t2259;
t2264 = t762.*t2235;
t2265 = t751.*t2237;
t2266 = t129.*t2252.*3.749399456654644e-33;
t2290 = t766.*t2248;
t2267 = -t819+t2254+t2255+t2264+t2265-t2290;
t2268 = t100.*t2250.*3.749399456654644e-33;
t2269 = t121.*t1803.*5.515;
t2270 = t520.*t806.*5.515;
t2271 = t2269+t2270;
t2272 = t95.*t2212;
t2273 = t121.*t2216;
t2274 = t15.*t930;
t2385 = t15.*t2219;
t2386 = t95.*t960;
t2275 = t2272+t2273+t2274-t2385-t2386;
t2297 = t13.*t2233.*2.152934142846781e-1;
t2276 = t142+t143+t144+t146+t465+t466+t467-t709+t2242-t2297;
t2277 = t124.*(t1129+t1130+t1131-t1976-t1977-t1978);
t2278 = t1128+t1132-t1975-t1979-t1980+t2277;
t2295 = t960.*t2233;
t2279 = t1026+t1027-t2295;
t2294 = t1004.*t2233;
t2280 = t1023+t1025-t2294;
t2283 = t121.*t416.*(3.49e2./2.0e2);
t2284 = t444.*t462.*(3.49e2./2.0e2);
t2285 = t2283+t2284;
t2286 = t95.*t1004;
t2287 = t15.*t2228;
t2288 = t121.*t2226;
t2394 = t15.*t1008;
t2395 = t95.*t2222;
t2289 = t2286+t2287+t2288-t2394-t2395;
t2296 = t120.*t2233.*3.749399456654644e-33;
t2298 = t121.*t2276.*5.515;
t2299 = t708+t2298;
t2301 = t121.*t2276;
t2302 = t1413+t2301;
t2303 = t101.*(t403+t404+t405-t833+t1056-t1851).*5.515;
t2304 = t142+t143+t648+t649+t650-t705-t706-t707+t2242-t2297;
t2305 = t11.*t2233.*2.152934142846781e-1;
t2306 = t13.*t2233.*9.274373618014111e-4;
t2307 = -t581+t712+t2305+t2306;
t2312 = t134.*t2233;
t2375 = t442.*t2250;
t2376 = t488.*t2252;
t2313 = t2120+t2121+t2123+t2312-t2375-t2376;
t2314 = t2233.*t2237;
t2315 = t1093.*t2250;
t2316 = t2210.*t2252;
t2317 = t2054.*t2235;
t2318 = t129.*t2050.*3.749399456654644e-33;
t2319 = t398.*t646.*3.749399456654644e-33;
t2320 = t772.*t2233;
t2321 = t788.*t2050;
t2322 = t646.*t1127;
t2323 = t780.*t2054;
t2430 = t2208.*t2250;
t2431 = t1136.*t2252;
t2324 = t2320+t2321+t2322+t2323-t2430-t2431;
t2325 = t100.*t2054.*3.749399456654644e-33;
t2326 = t2050.*t2248;
t2428 = t646.*t2207;
t2327 = t2314+t2315+t2316+t2317+t2326-t2428;
t2328 = t13.*t2233.*8.169842925973351e-1;
t2329 = t617-t1068+t2234+t2328;
t2330 = t11.*t2233.*4.876002456295764e-2;
t2331 = -t623+t1826+t2256+t2330;
t2332 = t11.*t2233.*8.979785040610579e-2;
t2333 = t13.*t2233.*1.139316919009596e-3;
t2334 = -t1064+t1824+t2332+t2333;
t2335 = t444.*t805;
t2336 = t392.*t2235;
t2337 = t164.*(t1094+t1095+t1096+t1097-t1862-t1863);
t2338 = t15.*t2237;
t2339 = t101.*(t1100+t1101+t1102+t1103-t1864-t1865);
t2344 = t456.*t2248;
t2340 = -t1861+t2336+t2337+t2338+t2339-t2344;
t2374 = t806.*t2276;
t2343 = t1962-t2374;
t2345 = t442.*t762.*3.749399456654644e-33;
t2346 = t734.*t772;
t2347 = t398.*t751.*3.749399456654644e-33;
t2348 = t134.*t734.*3.749399456654644e-33;
t2349 = t766.*t2210;
t2350 = t806.*t829.*5.515;
t2365 = t444.*t1803;
t2351 = t2206-t2365;
t2352 = t129.*(t2034-t2097);
t2353 = t2039+t2040+t2041-t2098-t2099+t2352;
t2354 = t734.*t2237;
t2355 = t788.*(t2034-t2097);
t2356 = t762.*(t1129+t1130+t1131-t1976-t1977-t1978);
t2387 = t13.*(t750-t754).*8.979785040610579e-2;
t2388 = t1124+t1125+t1126-t1900-t1901-t2387;
t2357 = t751.*t2388;
t2422 = t780.*t2038;
t2423 = t766.*t1136;
t2358 = t2346+t2355+t2356+t2357-t2422-t2423;
t2359 = t2209.*t2248;
t2419 = t762.*t1093;
t2420 = t751.*t2207;
t2421 = t2038.*t2235;
t2360 = t2349+t2354+t2359-t2419-t2420-t2421;
t2361 = t129.*t2209.*3.749399456654644e-33;
t2367 = t444.*t1803.*5.515;
t2362 = t2350-t2367;
t2373 = t806.*t2276.*5.515;
t2363 = t1866-t2373;
t2364 = (t727.*t2340)./2.0;
t2366 = t141+t142+t143+t144+t146+t147+t1435-t1496+t2242-t2297;
t2368 = (t57.*t2353)./2.0;
t2369 = t242.*t243.*7.02899814278107e-66;
t2370 = t388.*t2233;
t2371 = t2107+t2108-t2260+t2370-t242.*t2233;
t2372 = (t727.*t2371)./2.0;
t2380 = t948.*(t750-t754);
t2381 = t2130+t2131+t2132+t2133+t2380-t729.*t942;
t2382 = t727.*t2381;
t2383 = t2124+t2125+t2134+t2135+t2382-t366.*t758.*3.749399456654644e-33-t242.*t1532.*3.749399456654644e-33-t57.*t2129;
t2384 = (t57.*t2383)./2.0;
t2389 = (t1763.*t1764)./2.0;
t2390 = (t1768.*t1769)./2.0;
t2391 = t416.*t806.*(3.49e2./2.0e2);
t2392 = t2391-t444.*t993.*(3.49e2./2.0e2);
t2396 = (t57.*t2289)./2.0;
t2401 = t834.*t2233;
t2402 = t751.*t1852;
t2403 = t646.*t1853;
t2445 = t751.*t2304.*5.515;
t2404 = t1944-t2445;
t2585 = t734.*t2304;
t2405 = t2401+t2402+t2403-t2585;
t2406 = t834.*t2233.*5.515;
t2571 = t751.*t2304;
t2407 = t1987-t2571;
t2454 = t734.*t2304.*5.515;
t2408 = t2341+t2342+t2406-t2454;
t2409 = t603.*t2233;
t2410 = t15.*t2304;
t2436 = t101.*t2304.*5.515;
t2411 = t1063-t2436;
t2412 = t2169-t2300+t2409+t2410;
t2413 = t603.*t2233.*5.515;
t2414 = t15.*t2304.*5.515;
t2415 = -t1899+t2303+t2413+t2414;
t2536 = t101.*t2304;
t2416 = t1807-t2536;
t2443 = t101.*t2388;
t2417 = t1128+t1132-t1979-t1980+t2277-t2443;
t2418 = t121.*t2353;
t2424 = t806.*t2358;
t2425 = t444.*t2360;
t2426 = t2418+t2424+t2425;
t2427 = t121.*t2313;
t2429 = t444.*t2327;
t2432 = t2264+t2265-t2290;
t2433 = t11.*t2233.*5.114817050334782e-3;
t2532 = t13.*t2233.*1.18734317978;
t2434 = t179+t180+t181+t182+t183+t184+t185-t293+t2433-t2532;
t2456 = t121.*t2307;
t2435 = t2174-t2456;
t2439 = t129.*t2252;
t2440 = t100.*t2250;
t2441 = -t1138+t2439+t2440;
t2442 = t121.*t2441;
t2446 = t1397+t1398+t1399-t12.*t2276;
t2447 = t1293.*t2237;
t2448 = t1319.*t2235;
t2449 = t1314.*t2248;
t2450 = t1876+t1877-t1951+t2447+t2448+t2449;
t2451 = t806.*t2307;
t2452 = t2335+t2451;
t2581 = t57.*t2366.*5.515;
t2453 = t1583-t2581;
t2607 = t57.*t2366;
t2455 = t1588-t2607;
t2457 = t11.*t2233.*1.917749226941314e-35;
t2579 = t13.*t2233.*4.451823873129729e-33;
t2458 = t584+t585+t587+t588+t589+t591+t592+t1185-t1401+t2457-t2579;
t2459 = (t444.*t2340)./2.0;
t2460 = t667.*t2252;
t2461 = t1208.*t2237;
t2462 = t1330.*t2248;
t2463 = t660.*t2250;
t2464 = t1181.*t2250;
t2465 = t1166.*t2252;
t2466 = t1833+t1836-t1970+t1992+t2464+t2465;
t2467 = t286.*t2235;
t2468 = t425.*t2248;
t2469 = t530.*t2237;
t2470 = t661-t1416-t1417+t2467+t2468+t2469;
t2471 = t11.*t2233.*3.477333140419428e-36;
t2551 = t13.*t2233.*8.072210105402954e-34;
t2472 = t1296+t1297+t1298+t1299+t1300+t1301+t1303+t1304-t1353+t2471-t2551;
t2473 = (t806.*t2417)./2.0;
t2474 = t613.*t2252;
t2475 = t653.*t2250;
t2476 = t100.*t2252;
t2533 = t129.*t2250;
t2477 = -t2444+t2474+t2475+t2476-t2533;
t2478 = (t727.*t2477)./2.0;
t2479 = t1326.*t2235;
t2480 = -t1969+t2460+t2461+t2462+t2463+t2479;
t2481 = t1772+t1773-t1961-t729.*t2276;
t2482 = t100.*t164.*7.02899814278107e-66;
t2483 = t57.*t1822.*1.874699728327322e-33;
t2484 = t101.*t2334;
t2485 = t164.*t2235;
t2486 = t164.*t2329;
t2487 = t124.*t2248;
t2646 = t124.*t2331;
t2488 = t2484+t2485+t2486+t2487-t2646;
t2489 = t727.*t2488.*1.874699728327322e-33;
t2647 = t121.*t2307.*5.515;
t2490 = t1079-t2647;
t2491 = t646.*t2388;
t2492 = t2320+t2321+t2323-t2430-t2431+t2491;
t2493 = t806.*t2492;
t2494 = t101.*t598.*7.02899814278107e-66;
t2495 = t762.*t1820;
t2496 = t751.*t1813;
t2497 = t766.*t780;
t2498 = t762.*t788;
t2657 = t766.*t1816;
t2499 = t2495+t2496+t2497+t2498-t2657;
t2500 = t57.*t2499;
t2501 = t766.*t2235;
t2502 = t766.*t2329;
t2503 = t762.*t2248;
t2658 = t762.*t2331;
t2659 = t751.*t2334;
t2504 = t2501+t2502+t2503-t2658-t2659;
t2505 = t727.*t2504;
t2506 = t100.*t766.*3.749399456654644e-33;
t2507 = t613.*t766.*3.749399456654644e-33;
t2508 = t129.*t762.*3.749399456654644e-33;
t2660 = t653.*t762.*3.749399456654644e-33;
t2661 = t598.*t751.*3.749399456654644e-33;
t2509 = t2500+t2505+t2506+t2507+t2508-t2660-t2661;
t2510 = t806.*t2307.*5.515;
t2511 = t1953+t2510;
t2512 = t164.*t613.*7.02899814278107e-66;
t2513 = t124.*t129.*7.02899814278107e-66;
t2514 = t1816.*t2252;
t2515 = t788.*t2250;
t2516 = t1820.*t2250;
t2665 = t780.*t2252;
t2666 = t646.*t1813;
t2517 = t2514+t2515+t2516-t2665-t2666;
t2518 = t2235.*t2252;
t2519 = t2252.*t2329;
t2520 = t2250.*t2331;
t2668 = t2248.*t2250;
t2669 = t646.*t2334;
t2521 = t2518+t2519+t2520-t2668-t2669;
t2522 = t727.*t2521;
t2523 = t613.*t2252.*3.749399456654644e-33;
t2524 = t653.*t2250.*3.749399456654644e-33;
t2525 = t100.*t2252.*3.749399456654644e-33;
t2667 = t57.*t2517;
t2670 = t129.*t2250.*3.749399456654644e-33;
t2671 = t598.*t646.*3.749399456654644e-33;
t2526 = t2522+t2523+t2524+t2525-t2667-t2670-t2671;
t2527 = (t727.*t2526)./2.0;
t2528 = t2427+t2429+t2493;
t2529 = t444.*t2261;
t2530 = t806.*t2262;
t2531 = t2442+t2529+t2530;
t2534 = t444.*t2432;
t2535 = t1077+t1143+t2534;
t2537 = t11.*t2233.*1.18734317978;
t2538 = t13.*t2233.*5.114817050334782e-3;
t2539 = -t1156+t1295+t2537+t2538;
t2540 = t444.*t2267;
t2541 = t806.*t2261;
t2542 = t806.*t2263;
t2750 = t444.*t2262;
t2543 = t1077+t2540+t2541+t2542-t2750;
t2544 = t806.*t2267;
t2751 = t444.*t2263;
t2752 = t806.*t2432;
t2545 = t1147+t2442+t2544-t2751-t2752;
t2546 = (t805.*t1155)./2.0;
t2547 = t140+t141+t142+t143+t144+t146+t147-t205+t2242-t2297;
t2548 = (t827.*t1281)./2.0;
t2549 = (t100.*t164)./2.0;
t2550 = (t101.*t598)./2.0;
t2552 = (t164.*t613)./2.0;
t2553 = (t124.*t129)./2.0;
t2616 = t633.*t2252;
t2617 = t345.*t2250;
t2554 = t1324+t1327+t1331+t1332-t2616-t2617;
t2555 = (t1155.*t1575)./2.0;
t2556 = t727.*t2432;
t2557 = t1030+t1031+t1895-t2044+t2556;
t2558 = (t2302.*t2539)./2.0;
t2559 = (t57.*t2185)./2.0;
t2560 = t727.*t2267;
t2561 = t57.*t2261;
t2562 = t57.*t2263;
t2649 = t727.*t2262;
t2563 = t1030+t1031-t2044+t2560+t2561+t2562-t2649;
t2564 = t727.*t2261;
t2565 = t57.*t2262;
t2566 = -t1038+t2266+t2268+t2564+t2565;
t2567 = t57.*t2267;
t2568 = t124.*t653.*1.874699728327322e-33;
t2569 = (t1782.*t1911)./2.0;
t2570 = (t1155.*t2199)./2.0;
t2675 = t12.*t2276.*5.515;
t2572 = t843+t844+t1737-t2675;
t2573 = t57.*t1639;
t2574 = t129.*t164.*3.749399456654644e-33;
t2575 = t101.*t134.*3.749399456654644e-33;
t2576 = t164.*t2248;
t2577 = t101.*t2237;
t2612 = t124.*t2235;
t2578 = t2576+t2577-t2612;
t2580 = (t1742.*t1911)./2.0;
t2582 = (t2452.*t2453)./2.0;
t2583 = t57.*t2466;
t2584 = t727.*t2480;
t2586 = (t2435.*t2458)./2.0;
t2587 = (t806.*t2353)./2.0;
t2588 = (t1221.*t2180)./2.0;
t2589 = t11.*t2233.*4.451823873129729e-33;
t2590 = t13.*t2233.*1.917749226941314e-35;
t2591 = -t1200-t1604+t2011+t2589+t2590;
t2592 = (t1474.*t1629)./2.0;
t2593 = t57.*t2307.*5.515;
t2594 = t2188+t2593;
t2595 = (t2343.*t2594)./2.0;
t2596 = t727.*t2450;
t2597 = t1883+t1884+t1885+t1892+t1893-t2115-t2116+t2596;
t2598 = t530.*t2304;
t2599 = t1640-t2005-t2006+t2598;
t2679 = t633.*t2252.*3.749399456654644e-33;
t2680 = t345.*t2250.*3.749399456654644e-33;
t2600 = t1832+t1840+t1848+t1849+t2583+t2584-t2679-t2680;
t2684 = t729.*t2276.*5.515;
t2601 = t1777+t1778-t1857-t2684;
t2602 = (t1911.*t1919)./2.0;
t2603 = (t1221.*t2199)./2.0;
t2604 = t11.*t2233.*8.072210105402954e-34;
t2605 = t13.*t2233.*3.477333140419428e-36;
t2606 = -t1576-t1577+t1800+t2604+t2605;
t2608 = t1293.*t2304;
t2609 = t1867+t1868+t1870+t2608;
t2610 = t1293.*t2304.*5.515;
t2611 = t1963+t1964+t1965+t2610;
t2613 = t729.*t2262;
t2614 = t806.*t2466;
t2615 = t67.*t2261;
t2618 = t444.*t2477;
t2619 = t121.*t1205;
t2620 = t806.*t1639;
t2621 = t67.*t2432;
t2622 = t444.*t2450;
t2623 = t1998+t2001+t2002-t2171+t2621+t2622;
t2624 = t101.*t805;
t2625 = t640.*t751;
t2626 = t2624+t2625;
t2627 = t101.*t2307;
t2628 = t100.*t164;
t2629 = t101.*t598;
t2630 = t164.*t613;
t2631 = t124.*t129;
t2705 = t124.*t653;
t2632 = t2628+t2629+t2630+t2631-t2705;
t2633 = t121.*t2632;
t2634 = t530.*t2304.*5.515;
t2635 = t640.*t646;
t2636 = t2627+t2635;
t2637 = t444.*t2480;
t2638 = t121.*t2554;
t2739 = t12.*t2441;
t2639 = t2613+t2614+t2615+t2637+t2638-t2739;
t2640 = t1609-t1971-t1972+t2634;
t2641 = (t359.*t2416)./2.0;
t2642 = (t827.*t1629)./2.0;
t2643 = (t1265.*t1911)./2.0;
t2644 = (t2434.*t2599)./2.0;
t2645 = (t805.*t1221)./2.0;
t2648 = (t444.*t2557)./2.0;
t2650 = (t2028.*t2416)./2.0;
t2651 = -t1038+t2045+t2266+t2268+t2567-t57.*t2432-t727.*t2263;
t2652 = (t806.*t2651)./2.0;
t2653 = (t1115.*t1474)./2.0;
t2654 = (t878.*t2180)./2.0;
t2655 = (t2302.*t2490)./2.0;
t2656 = (t2299.*t2435)./2.0;
t2662 = (t57.*t2509)./2.0;
t2663 = (t2363.*t2452)./2.0;
t2664 = (t2343.*t2511)./2.0;
t2672 = t124.*t653.*7.02899814278107e-66;
t2673 = (t2165.*t2416)./2.0;
t2674 = (t2166.*t2407)./2.0;
t2676 = t727.*t2578;
t2677 = t2573+t2574+t2575+t2676-t100.*t124.*3.749399456654644e-33;
t2678 = (t727.*t2488)./2.0;
t2681 = (t444.*t2600)./2.0;
t2682 = (t67.*t2566)./2.0;
t2683 = (t2405.*t2453)./2.0;
t2685 = (t2407.*t2601)./2.0;
t2686 = t727.*t2470;
t2687 = t1921+t1922+t1930+t1933+t1934+t1941+t2686-t124.*t345.*3.749399456654644e-33;
t2688 = t57.*t2307;
t2689 = t1968+t2688;
t2690 = (t806.*t2597)./2.0;
t2691 = (t878.*t1575)./2.0;
t2692 = (t729.*t2557)./2.0;
t2693 = t646.*t805;
t2694 = (t2404.*t2405)./2.0;
t2695 = (t2407.*t2408)./2.0;
t2696 = t101.*(t403+t404+t405-t833+t1056-t1851);
t2697 = -t2300+t2409+t2410+t2696;
t2698 = (t2415.*t2416)./2.0;
t2699 = t121.*t1084;
t2700 = t444.*t2340;
t2701 = t806.*t2417;
t2702 = t2699+t2700+t2701;
t2703 = (t806.*t2426)./2.0;
t2706 = t751.*t2307;
t2704 = t2693-t2706;
t2707 = t646.*t805.*5.515;
t2708 = t806.*t2499;
t2709 = t444.*t2504;
t2710 = t121.*t2185;
t2711 = t2708+t2709+t2710;
t2712 = (t121.*t2702)./2.0;
t2713 = t101.*t805.*5.515;
t2714 = t640.*t751.*5.515;
t2715 = t2713+t2714;
t2716 = (t1110.*t2199)./2.0;
t2717 = (t1911.*t1956)./2.0;
t2718 = t444.*t2521;
t2719 = t121.*t2477;
t2720 = t2718+t2719-t806.*t2517;
t2721 = t101.*t2307.*5.515;
t2722 = t100.*t164.*3.749399456654644e-33;
t2723 = t57.*t1822;
t2724 = t727.*t2488;
t2725 = t101.*t598.*3.749399456654644e-33;
t2726 = t164.*t613.*3.749399456654644e-33;
t2727 = t124.*t129.*3.749399456654644e-33;
t2728 = t2722+t2723+t2724+t2725+t2726+t2727-t124.*t653.*3.749399456654644e-33;
t2729 = (t444.*t2528)./2.0;
t2733 = t751.*t2307.*5.515;
t2730 = t2707-t2733;
t2731 = t640.*t646.*5.515;
t2732 = t2721+t2731;
t2734 = (t729.*t2535)./2.0;
t2735 = (t49-t63-t64+t137+t138-t642).*(t964+t965+t966-t1222+t1291-t1584-t1585-t1586);
t2736 = t1867+t1868+t2608+t2735;
t2737 = t444.*t2470;
t2738 = t2008+t2010+t2017+t2737-t729.*t1639-t67.*t2578;
t2740 = t444.*t2578;
t2741 = t2619+t2620+t2740;
t2742 = (t806.*t2623)./2.0;
t2743 = (t67.*t2531)./2.0;
t2744 = (t444.*t2639)./2.0;
t2745 = (t2411.*t2599)./2.0;
t2746 = (t2416.*t2640)./2.0;
t2747 = (t806.*t1822)./2.0;
t2748 = (t444.*t2535)./2.0;
t2749 = (t444.*t2488)./2.0;
t2753 = (t806.*t2545)./2.0;
t2754 = (t806.*t2185)./2.0;
C = reshape([qd2.*(t2.*(-1.141223459619257e-35)-t3.*5.504493342314691e-37+t241+t252+t255+t266+t276+t284+t304+t310+t322+t336+t346+t353+t360+t367+t375+t384+(t162.*(t234+t236+t237-t3.*t22.*2.206-t8.*t34.*6.053757698066069e-1-t13.*t44.*1.18734317978+t11.*(t37+t41-t3.*t22-t8.*t34.*6.123233995736766e-17).*1.18734317978+t13.*(t37+t41-t3.*t22-t8.*t39.*6.123233995736766e-17).*5.114817050334782e-3))./2.0-(t12.*t215)./2.0-(t129.*t218)./2.0-(t12.*t338)./2.0-(t100.*t286)./2.0-(t7.*t381)./2.0-(t164.*t233)./2.0-(t101.*t317)./2.0-(t121.*t379)./2.0+(t292.*(t20.*(-1.0616375)+t179+t180+t181+t182+t183+t184+t185-t11.*t84.*5.114817050334782e-3+t13.*t84.*1.18734317978))./2.0-(t243.*(t2.*(-2.033158615944436e-19)+t88+t112+t113+t115-t6.*t12.*4.4101e-6-7.623123809914776e-52))./2.0-(t134.*(t5+t9+t80-t6.*t10))./2.0)+qd4.*(t654+t1150+t1160-(t124.*t129)./2.0-(t100.*t164)./2.0-(t101.*t598)./2.0-(t164.*t613)./2.0+(t195.*t692)./2.0+(t162.*(t11.*t53.*5.114817050334782e-3-t13.*t53.*1.18734317978+t11.*t56.*1.18734317978+t13.*t56.*5.114817050334782e-3))./2.0)+qd3.*(t393+t400+t412+t422+t437+t443+t475+t984+t989+t994+t996+(t94.*(t6.*t45.*2.6117415e-2+t8.*t45.*2.799678e-4-t6.*t48.*2.799678e-4+t8.*t48.*2.6117415e-2))./2.0-(t15.*t388)./2.0-(t101.*t398)./2.0-(t129.*t456)./2.0-(t164.*t488)./2.0+(t170.*t492)./2.0+(t195.*t501)./2.0+(t162.*(t6.*t45.*6.053757698066069e-1+t8.*t48.*6.053757698066069e-1+t11.*t150.*5.114817050334782e-3-t13.*t150.*1.18734317978+t11.*t153.*1.18734317978+t13.*t153.*5.114817050334782e-3))./2.0),qd4.*(t654-t1199-t1206+t1582+t1624+t1625+t1982+t1984+t1986+t2555-(t124.*t129)./2.0-(t100.*t164)./2.0-(t101.*t598)./2.0-(t164.*t613)./2.0+(t359.*t1590)./2.0-(t197.*t1910)./2.0-(t1265.*t1911)./2.0+(t1305.*(t1156+t1157+t1158-t1295))./2.0+(t444.*(t1324+t1327+t1331+t1332-t345.*t775-t633.*t783))./2.0)+qd2.*(t2.*(-2.282446919238515e-35)-t3.*1.100898668462938e-36-t1193-t1194-t1195-t1196-t1197+t1270+t120.*(t29+t30)-t12.*t215+t12.*t309+t15.*t321-t12.*t338-t7.*t381+t95.*t366-t242.*t243-t121.*t379+t281.*t1369+t359.*t1305+t177.*t1507+t197.*t1488+t270.*t1662+t303.*t1682+t1155.*t1390+t1265.*t1290+t1251.*t1349+t1227.*t1412-t1254.*t1657+t1252.*t1677+t240.*(t3-t5))+qd1.*(t2.*(-1.141223459619257e-35)-t3.*5.504493342314691e-37+t241+t255+t276+t284+t304+t310+t322+t346+t360+t367+t375+t1234+(t1254.*(t221+t222+t223-t1223-t2.*t727.*2.6811e-2-t3.*t727.*3.0849e-3))./2.0-(t12.*t215)./2.0-(t12.*t338)./2.0-(t100.*t286)./2.0-(t7.*t381)./2.0-(t242.*t243)./2.0-(t121.*t379)./2.0-(t129.*t425)./2.0-(t134.*t530)./2.0-(t101.*t636)./2.0-(t164.*t633)./2.0+(t827.*t1265)./2.0+(t851.*t1251)./2.0+(t1155.*t1190)./2.0+(t1225.*t1227)./2.0+(t1252.*t1666)./2.0)+qd3.*(t393+t400+t412+t422+t437+t443+t475-t848-t852-t885-t909-t910-t973+t1394+t1396+t1783+t1784+t1786+t1788+t1789+t1790+t1791+t1792+t1794+t1796+t1798+t1799+t2069+t2070+t2071+t2072+t2073+t2074+t2075+t2079+t2080-(t15.*t388)./2.0-t242.*t243.*1.874699728327322e-33-(t101.*t398)./2.0-(t129.*t456)./2.0-(t164.*t488)./2.0-(t57.*t1537)./2.0-(t727.*t1544)./2.0),-qd4.*(t1062-t1085+t1086+t1087+t1112+t2022+t2027+t2177+t2197+t2198+t2569+t2570-t124.*t653.*1.874699728327322e-33-(t57.*t1140)./2.0-(t57.*t2185)./2.0-(t197.*t2170)./2.0-(t197.*t2175)./2.0-(t1159.*t1415)./2.0-(t727.*t2024)./2.0-(t1281.*t1474)./2.0-(t1155.*t2180)./2.0-(t1590.*t2028)./2.0)+qd1.*(t393+t400+t412+t422+t437+t443+t475+t984+t994+t2029+t2030-(t15.*t388)./2.0-(t101.*t398)./2.0-(t129.*t456)./2.0-(t164.*t488)./2.0+(t827.*t1782)./2.0+(t1155.*t1803)./2.0+(t197.*(t403+t404+t405+t406-t833-t853))./2.0+(t148.*(t985+t986+t987+t988-t1351-t1352))./2.0)+qd3.*(-t2047-t2060-t2063-t2068+t2088+t2095+t2100+t2112+t2114+t2117+t2137+t2145-t15.*t388.*3.749399456654644e-33-t101.*t398.*3.749399456654644e-33-t129.*t456.*3.749399456654644e-33-t164.*t488.*3.749399456654644e-33+(t57.*t1036)./2.0-t57.*t2042+t177.*t2094+t197.*t2103+t983.*t1467+t1343.*t1378-t727.*t2056-t727.*t2110+t1474.*t1782+t1155.*t2106+t1227.*t2091+(t727.*(t1029+t1030+t1031+t1033+t2043-t2044-t727.*t814))./2.0+t1415.*(t985+t986+t987+t988-t1351-t1352)+(t57.*(t1055+t2061+t2062-t139.*t242.*3.749399456654644e-33-t309.*t444.*3.749399456654644e-33))./2.0+(t727.*(t1039+t1040+t2033-t309.*t806.*3.749399456654644e-33-t727.*t1046-t57.*t2031+t727.*t2032))./2.0)+qd2.*(t393+t400+t412+t422+t437+t443+t475-t848-t852-t885-t909-t910-t973+t1394+t1783+t1786+t1788+t1789+t1790+t1791+t1792+t1794+t1796+t1798+t1799+t2069+t2070+t2071+t2072+t2073+t2074+t2075+t2079+t2080+(t197.*(t1460+t1461+t1462+t1463+t1464-t1872-t1873))./2.0-(t15.*t388)./2.0-t242.*t243.*1.874699728327322e-33-(t101.*t398)./2.0-(t129.*t456)./2.0-(t164.*t488)./2.0-(t57.*t1537)./2.0-(t727.*t1544)./2.0+(t727.*(t1324+t1327+t1331+t1332-t1606-t1607))./2.0),-qd1.*(-t654-t2546-t2548+t2549+t2550+t2552+t2553+(t2307.*t2434)./2.0+(t2539.*t2547)./2.0)-qd3.*(t1062-t1085+t1086+t1087+t1112+t2478+t2558-t2559-t2568+t2569+t2570+t2587+t2648+t2650+t2652-(t1281.*t1474)./2.0-(t444.*t2313)./2.0-(t444.*t2563)./2.0-(t1155.*t2180)./2.0-(t806.*t2566)./2.0-(t2412.*t2434)./2.0-(t2434.*t2435)./2.0)-qd2.*(-t654+t1199+t1206-t1582-t1625-t1982-t1984+t2549+t2550+t2552+t2553-t2555+t2641+t2643+t2644-(t67.*t2441)./2.0-(t444.*t2554)./2.0+(t2472.*t2539)./2.0+(t2434.*t2606)./2.0)-qd4.*(t2618+t2633+t2748+t2753-(t444.*t2543)./2.0-t806.*t2185+t1281.*t1911-(t806.*t2531)./2.0-t1155.*t2626-t2416.*t2539+t2434.*t2636),qd4.*(t654+t1199+t1206-(t45.*(t101.*t565-t124.*t545+t164.*t555))./2.0+(t162.*(t1184+t11.*t53.*1.917749226941314e-35-t13.*t53.*4.451823873129729e-33+t11.*t56.*4.451823873129729e-33+t13.*t56.*1.917749226941314e-35))./2.0-(t162.*(t603.*(t35-t40-t6.*t36+t8.*t39).*5.515+t530.*t609.*5.515+t610.*t647.*5.515+t101.*(t348+t349+t350-t432-t2.*t20.*2.540928714850161e-34+t3.*t22.*4.149651502162508e-18+t6.*t36.*6.776895191416263e-2-t8.*t39.*6.776895191416263e-2).*5.515))./2.0-(t124.*t129)./2.0-(t100.*t164)./2.0-(t101.*t598)./2.0-(t164.*t613)./2.0-(t292.*t714)./2.0+(t427.*t580)./2.0+(t692.*t703)./2.0+(t148.*(t1200+t1201+t1202-t13.*t78.*4.451823873129729e-33-t22.*t640.*5.515))./2.0-(t67.*(t1191+t1192-t124.*t620))./2.0+(t593.*(t20.*(-2.946606165491677e-33)+t584+t585+t587+t588+t589+t590+t591+t592-t11.*t84.*1.917749226941314e-35-t22.*t586.*5.515))./2.0+(t148.*(t1214+t646.*t647.*5.515-t101.*t1211.*5.515-t603.*t1208.*5.515))./2.0+(t444.*(t661+t682+t870+t871-t101.*t681-t164.*t667))./2.0+(t352.*(t101.*t609.*5.515-t603.*t610.*5.515))./2.0)-qd1.*(t2.*(-1.141223459619257e-35)-t3.*5.504493342314691e-37+t241+t252+t255+t266+t276+t284+t304+t310+t322+t336+t346+t353+t360+t367+t375+t384+t1234-(t12.*t215)./2.0-(t129.*t218)./2.0-(t12.*t338)./2.0-(t100.*t286)./2.0-(t7.*t381)./2.0-(t164.*t233)./2.0-(t101.*t317)./2.0-(t242.*t243)./2.0-(t121.*t379)./2.0-(t134.*t426)./2.0+(t162.*(t234+t236+t237-t3.*t22.*2.206-t8.*t39.*6.053757698066069e-1-t13.*t44.*1.18734317978+t11.*t81.*1.18734317978+t13.*t81.*5.114817050334782e-3))./2.0)+qd3.*(t393+t400+t412+t422+t437+t443+t475+t848+t852+t862+t885+t909+t910+t973+(t148.*(t969+t970+t971+t972-t8.*t65.*2.269795582384779e-33-t13.*t139.*4.451823873129729e-33-t520.*(t20-t23).*5.515))./2.0-(t162.*(t121.*(t348+t349+t350+t351-t430-t432+t962-t3.*t22.*2.6e-1).*5.515+t45.*t429.*5.515-t12.*t512.*5.515+t427.*t514.*5.515))./2.0+(t492.*(t917+t918+t920+t921-t6.*t45.*1.049711117200796e-36+t8.*t45.*9.792462161022385e-35-t6.*t48.*9.792462161022385e-35-t8.*t48.*1.049711117200796e-36+t2.*(t20-t23).*1.804608079944675e-33))./2.0-(t94.*(t121.*(t245+t246+t247-t385+t836-t3.*t22.*1.3582e-1).*(3.49e2./2.0e2)-t12.*t483.*(3.49e2./2.0e2)+t45.*t450.*(3.49e2./2.0e2)+t427.*t453.*(3.49e2./2.0e2)))./2.0+(t94.*(t850+t6.*t45.*9.792462161022385e-35+t8.*t45.*1.049711117200796e-36-t6.*t48.*1.049711117200796e-36+t8.*t48.*9.792462161022385e-35))./2.0-t31.*t120.*1.874699728327322e-33-t12.*t309.*1.874699728327322e-33-t15.*t321.*1.874699728327322e-33-(t15.*t388)./2.0-t95.*t366.*1.874699728327322e-33-t124.*t345.*1.874699728327322e-33-(t101.*t398)./2.0-(t129.*t456)./2.0+(t57.*t580)./2.0-(t164.*t488)./2.0-(t22.*t961)./2.0-(t148.*t847)./2.0-(t292.*t711)./2.0-(t111.*t905)./2.0+(t501.*t703)./2.0-(t372.*t976)./2.0+(t162.*(t887+t6.*t45.*2.269795582384779e-33+t8.*t48.*2.269795582384779e-33+t11.*t150.*1.917749226941314e-35-t13.*t150.*4.451823873129729e-33+t11.*t153.*4.451823873129729e-33+t13.*t153.*1.917749226941314e-35))./2.0+(t416.*(t20.*(-9.323350423903855e-34)+t855+t856+t857+t858+t860+t861-t22.*(t2.*(-1.688910400704115e-17)+t417+t418+t419+t493-t6.*t12.*1.6044e-4-5.342894225732868e-34).*(3.49e2./2.0e2)-t6.*t67.*1.049711117200796e-36))./2.0-(t22.*(t661+t682+t426.*(t20.*(-2.881087492837848e-33)+t626+t627+t628+t629+t630-t6.*t65.*7.684130555159526e-1-t8.*t67.*7.684130555159526e-1-t11.*t84.*1.139316919009596e-3+t13.*t84.*8.979785040610579e-2)-t101.*t681-t164.*t667+t425.*(t20.*(-4.271754237092021e-36)+t621+t622+t623+t624+t625+t719-t6.*t65.*1.139316919009596e-3-t8.*t67.*1.139316919009596e-3-t11.*t84.*8.169842925973351e-1)))./2.0+(t829.*(t20.*(-2.946606165491677e-33)+t584+t585+t587+t588+t589+t590+t591+t592-t11.*t84.*1.917749226941314e-35-t22.*(t2.*(-2.449293598294706e-17)+t407+t408+t409+t410+t411+t502-t11.*t15.*9.274373618014111e-4-5.342894225732869e-34).*5.515))./2.0-(t248.*(t121.*t483.*(3.49e2./2.0e2)+t427.*t450.*(3.49e2./2.0e2)))./2.0-(t352.*(t121.*t512.*5.515+t427.*t429.*5.515))./2.0+(t111.*(t906+t907+t908-t8.*t65.*9.792462161022385e-35-t22.*t462.*(3.49e2./2.0e2)))./2.0-(t57.*(t243.*(t892+t893+t894+t2.*t22.*3.3204e-3-t6.*t45.*4.4101e-6+t8.*t45.*2.53e-2-t6.*t48.*2.53e-2-t8.*t48.*4.4101e-6)+t31.*(t889+t890+t891+t2.*t22.*1.4955e-5+t6.*t45.*2.5506e-2-t8.*t45.*4.4101e-6+t6.*t48.*4.4101e-6+t8.*t48.*2.5506e-2)-t95.*(t898-t3.*t22.*3.3204e-3+t6.*t36.*2.53e-2+t8.*t36.*4.4101e-6+t6.*t39.*4.4101e-6-t8.*t39.*2.53e-2)-t121.*(t2.*t20.*(-2.092860147402869e-19)+t3.*t22.*3.4179e-3-t6.*t36.*3.3204e-3+t8.*t36.*1.4955e-5+t6.*t39.*1.4955e-5+t8.*t39.*3.3204e-3)+t15.*(t2.*t20.*(-9.157296440624334e-22)+t3.*t22.*1.4955e-5+t6.*t36.*4.4101e-6+t8.*t36.*2.5506e-2+t6.*t39.*2.5506e-2-t8.*t39.*4.4101e-6)-t12.*(t895+t896+t897+t6.*t45.*1.4955e-5+t8.*t45.*3.3204e-3-t6.*t48.*3.3204e-3+t8.*t48.*1.4955e-5+t2.*(t20-t23).*3.4179e-3)))./2.0),qd2.*(t2.*(-1.141223459619257e-35)-t3.*5.504493342314691e-37+t241+t255+t310+t322+t346+t367+((t57.*t298-t727.*t1666).*(t57.*t1669.*(9.01e2./2.0e2)-t727.*t1672.*(9.01e2./2.0e2)))./2.0+((t57.*t1669-t727.*t1672).*(t57.*t298.*(9.01e2./2.0e2)-t727.*t1666.*(9.01e2./2.0e2)))./2.0-(t12.*t215)./2.0-(t12.*t338)./2.0-(t100.*t286)./2.0-(t7.*t381)./2.0-(t242.*t243)./2.0-(t121.*t379)./2.0-(t129.*t425)./2.0-(t134.*t530)./2.0-(t101.*t636)./2.0-(t164.*t633)./2.0+(t1221.*t1390)./2.0+(t1186.*t1488)./2.0+(t1305.*t1597)./2.0+(t1290.*t1619)./2.0+(t1412.*t1521)./2.0+(t1349.*t1648)./2.0+(t1495.*t1507)./2.0+(t1369.*t1688)./2.0+(t1421.*t1694)./2.0+(t1424.*t1691)./2.0+(t1498.*t1623)./2.0+(t1500.*t1621)./2.0+(t1662.*t1719)./2.0-(t1657.*t1727)./2.0-(t1677.*t1710)./2.0+(t1682.*t1735)./2.0)+qd1.*((t1727.*(t221+t222+t223-t1223-t1728-t1729))./2.0+(t292.*t1186)./2.0-(t281.*t1369)./2.0-(t359.*t1305)./2.0-(t177.*t1507)./2.0-(t197.*t1488)./2.0+(t148.*t1597)./2.0+(t111.*t1688)./2.0+(t372.*t1495)./2.0-(t270.*t1662)./2.0-(t303.*t1682)./2.0+(t275.*t1719)./2.0+(t298.*t1735)./2.0+(t1190.*t1221)./2.0+(t827.*t1619)./2.0+(t851.*t1648)./2.0-(t1155.*t1390)./2.0-(t1265.*t1290)./2.0-(t1251.*t1349)./2.0-(t1227.*t1412)./2.0+(t1225.*t1521)./2.0+(t1254.*t1657)./2.0-(t1252.*t1677)./2.0-(t1666.*t1710)./2.0)+qd3.*(t393+t400+t412+t422+t437+t443+t475+t1394+t1396+t1418+t1459+t1531+t1553+t1914+t1917+t1920+t1927+t1929+t1932+t1935+t1936+t1937+t1938-(t15.*t388)./2.0-(t101.*t398)./2.0-(t129.*t456)./2.0-(t164.*t488)./2.0-(t57.*t1537)./2.0-(t711.*t1488)./2.0-(t878.*t1390)./2.0-(t727.*t1544)./2.0-(t976.*t1507)./2.0+(t1186.*t1400)./2.0+(t1221.*t1478)./2.0-(t1405.*t1412)./2.0+(t1415.*t1597)./2.0+(t1378.*t1648)./2.0-(t1290.*t1742)./2.0-(t1305.*t1738)./2.0+(t1495.*t1557)./2.0+(t1521.*t1564)./2.0+(t1474.*t1619)./2.0-(t1349.*t1746)./2.0-(t1369.*t1749)./2.0+(t1467.*t1688)./2.0-(t1421.*t1764)./2.0+(t1424.*t1769)./2.0-(t1498.*t1774)./2.0+(t1500.*t1779)./2.0-(t1623.*t1771)./2.0+(t1621.*t1776)./2.0-(t1694.*t1763)./2.0+(t1691.*t1768)./2.0+(t1498.*(t1804-t727.*t977))./2.0+(t1186.*(t1460+t1461+t1462+t1463+t1464-t8.*t65.*4.115676486645111e-34-t13.*t139.*8.072210105402954e-34))./2.0)+qd4.*(t654+t1581+t1582+t1624+t1625+t1630+t2007+t2009+t2012+t2013+t2016+t2019-(t124.*t129)./2.0-(t100.*t164)./2.0-(t101.*t598)./2.0-(t164.*t613)./2.0-(t67.*t1603)./2.0+(t444.*t1608)./2.0-(t714.*t1488)./2.0-(t729.*t1639)./2.0+(t1110.*t1390)./2.0+(t1221.*t1575)./2.0+(t1305.*t1610)./2.0-(t1186.*t1910)./2.0+(t1590.*t1597)./2.0-(t1290.*t1974)./2.0+(t1498.*t1871)./2.0-(t1623.*t1806)./2.0-(t1500.*t1967)./2.0+(t1621.*t1855)./2.0-(t1619.*t1911)./2.0),qd3.*(t2087+t2088+t2095+t2096+t2100+t2112+t2113+t2114+t2117+t2118+t2119+t2136+t2137+t2140+t2145+t2148+t2149+t2164+t2384+(t727.*(t2154+t2155+t2156+t2157+t2158-t242.*t1538.*3.749399456654644e-33-t57.*t2163+t321.*(t79-t85).*3.749399456654644e-33))./2.0+t1415.*(t969+t970+t971+t972+t1501-t2085-t2086)-(t727.*(t1832+t1840+t1848+t1849-t2146-t2147+t57.*t1993+t727.*t1990))./2.0-t31.*t120.*7.02899814278107e-66-t12.*t309.*7.02899814278107e-66-t15.*t321.*7.02899814278107e-66-t15.*t388.*3.749399456654644e-33-t95.*t366.*7.02899814278107e-66-t124.*t345.*7.02899814278107e-66-t101.*t398.*3.749399456654644e-33-t129.*t456.*3.749399456654644e-33-t164.*t488.*3.749399456654644e-33-(t57.*t1894)./2.0-t57.*t2042-(t711.*t1400)./2.0-(t878.*t1478)./2.0-(t976.*t1557)./2.0-t727.*t2056-t727.*t2110+t1378.*t1471+t1441.*t1467-(t1405.*t1564)./2.0-(t1378.*t1746)./2.0-(t1415.*t1738)./2.0-(t1467.*t1749)./2.0-(t1474.*t1742)./2.0+t1186.*t2103+t1221.*t2106+t1474.*t1919+t1495.*t2094+t1521.*t2091+t1421.*t2205+t1498.*t2351+t242.*(t80-t323).*7.02899814278107e-66+t1776.*(t1926-t2084)+t1916.*(t1765-t2111)+(t1776.*(t1777+t1778-t1856-t1857))./2.0+(t1771.*(t1772+t1773-t1960-t1961))./2.0+((t1765-t2111).*(t1766+t1767-t1924-t1925))./2.0+((t1760-t1939).*(t1761+t1762-t2138-t2139))./2.0)+qd1.*(t393+t400+t412+t422+t437+t443+t475+t848+t852+t862+t885+t909+t910+t973-t1394-t1396-t1790-t1791-t1792-t1796-t2069-t2071-t2072-t2073-t2074-t2075-t2079-t2080+t2200+t2201+t2202+t2203+(t148.*(t969+t970+t971+t972+t1501-t2085-t2086))./2.0-t31.*t120.*1.874699728327322e-33-(t15.*t388)./2.0-(t101.*t398)./2.0-(t129.*t456)./2.0-(t164.*t488)./2.0+(t57.*t1537)./2.0+(t827.*t1919)./2.0+(t1221.*t1803)./2.0+(t727.*(t1539+t1540+t1541+t1542-t2078+t321.*(t79-t85)))./2.0+(t1186.*(t403+t404+t405+t406-t833-t853))./2.0)+qd2.*(t393+t400+t412+t422+t437+t443+t475+t1914+t1917+t1920+t1927+t1929+t1932+t1935+t1936+t1937+t1938+(t1186.*(t1460+t1461+t1462+t1463+t1464-t1872-t1873))./2.0-(t15.*t388)./2.0-(t101.*t398)./2.0-(t129.*t456)./2.0-(t164.*t488)./2.0+(t1498.*(t1804-t1943))./2.0)-qd4.*(t1062-t1085+t1086+t1087+t1112+t2167+t2172+t2176+t2177+t2181+t2190+t2191+t2192+t2197+t2198+t2602+t2603-t124.*t653.*1.874699728327322e-33-t12.*t1205.*1.874699728327322e-33-t121.*t1198.*1.874699728327322e-33-t444.*t1216.*1.874699728327322e-33-t806.*t1183.*1.874699728327322e-33-(t57.*t2185)./2.0-(t1110.*t1478)./2.0-(t1415.*t1605)./2.0-(t1415.*t1610)./2.0-(t1474.*t1629)./2.0-(t1186.*t2170)./2.0-(t1186.*t2175)./2.0-(t1221.*t2180)./2.0-(t1774.*t1806)./2.0-(t1590.*t2165)./2.0-(t1776.*t2015)./2.0-(t1855.*t2166)./2.0+(t1498.*(t84.*t834+t651.*t734-t646.*t1853-t751.*t1852))./2.0+(t1498.*(t2335-t593.*t806))./2.0),-qd1.*(-t654-t1199-t1206+t1582+t1625+t2549+t2550+t2552+t2553+t2555-t2641-t2642-t2643-t2644-t2645+(t67.*t2441)./2.0+(t444.*t2554)./2.0+(t2307.*t2458)./2.0+(t2547.*t2591)./2.0)-qd4.*(t2618+t2633+t2734+t2742+t2743+t2744+t2745+t2746-(t1110.*t1575)./2.0-(t12.*t2741)./2.0-(t121.*t2738)./2.0-t806.*t2185+t1629.*t1911-t1221.*t2626-(t1911.*t1974)./2.0-t2407.*t2594-t2416.*t2591-(t2404.*t2609)./2.0-(t2407.*t2611)./2.0+t2458.*t2636+t2453.*t2704)-qd3.*(t1062-t1085+t1086+t1087+t1112+t2478-t2559-t2568-t2580-t2582-t2586+t2587-t2588-t2592-t2595+t2602+t2603+t2673+t2674+t2681+t2682+t2683+t2685+t2690+t2691+t2692-(t12.*t2677)./2.0-(t444.*t2313)./2.0-(t121.*t2687)./2.0-(t2412.*t2458)./2.0+(t2302.*t2591)./2.0-(t2299.*t2599)./2.0-(t2363.*t2609)./2.0-(t2416.*t2572)./2.0)-qd2.*(-t654-t2009-t2019+t2549+t2550+t2552+t2553-(t2455.*t2594)./2.0+(t2472.*t2591)./2.0+(t2458.*t2606)./2.0-(t2453.*t2689)./2.0),qd3.*(t2047+t2060+t2063+t2068-(t57.*t1036)./2.0-(t727.*(t1029+t1030+t1031+t1033+t2043-t129.*t766.*3.749399456654644e-33-t727.*t814))./2.0-(t57.*(t1055+t2061+t2062-t139.*t242.*3.749399456654644e-33-t309.*t444.*3.749399456654644e-33))./2.0-(t727.*(t1039+t1040+t2033-t309.*t806.*3.749399456654644e-33-t727.*t1046-t57.*(t1026+t1027+t1043+t1054-t734.*t1004-t806.*t1012)+t727.*(t1023+t1024+t1025+t1041+t1042-t758.*t930)))./2.0)-qd1.*(t393+t400+t412+t422+t437+t443+t475+t984+t989+t994+t996+t2029+t2030-(t15.*t388)./2.0-(t101.*t398)./2.0-(t129.*t456)./2.0-(t164.*t488)./2.0+(t977.*t1155)./2.0+(t827.*(t1333+t1334+t1335+t1336-t11.*t758.*5.114817050334782e-3+t13.*t758.*1.18734317978))./2.0)-qd4.*(t1061+t1062+t1085+t1086+t1087+t1106+t1112+(t444.*(t1029+t1030+t1031+t1033+t57.*t831-t129.*t766.*3.749399456654644e-33-t727.*t814))./2.0-(t444.*(t57.*(t545.*t725+t565.*t722+t555.*t741)+t727.*(t767+t620.*t762-t673.*t766)+t100.*t725.*3.749399456654644e-33+t134.*t722.*3.749399456654644e-33+t129.*t741.*3.749399456654644e-33))./2.0-(t806.*(t818+t820+t1037-t134.*t646.*3.749399456654644e-33-t727.*t831-t57.*(t767+t817-t673.*t766)+t727.*(t815+t816-t766.*t788)))./2.0-t124.*t653.*1.874699728327322e-33-(t148.*t1080)./2.0-(t593.*t711)./2.0+(t714.*t829)./2.0-(t805.*t878)./2.0+(t806.*t1036)./2.0-(t827.*t1115)./2.0-(t977.*t1110)./2.0+(t57.*(t124.*t555+t164.*t545+t124.*(t551+t553-t13.*t53.*4.876002456295764e-2+t11.*t56.*4.876002456295764e-2)-t164.*(-t542+t686+t11.*t53.*8.169842925973351e-1+t13.*t56.*8.169842925973351e-1)-t101.*(t11.*t53.*1.139316919009596e-3-t13.*t53.*8.979785040610579e-2+t11.*t56.*8.979785040610579e-2+t13.*t56.*1.139316919009596e-3)))./2.0-(t827.*(t1120+t1121-t751.*t823.*5.515-t101.*(t825+t826+t828+t1122+t1123-t11.*t758.*9.274373618014111e-4).*5.515))./2.0+(t806.*(t1128+t1132-t101.*t1127-t456.*t788-t164.*t1136+t124.*(t1129+t1130+t1131-t11.*t757.*4.876002456295764e-2-t13.*t757.*2.53401226709415e-4-t13.*t758.*4.876002456295764e-2)))./2.0-(t22.*(t1071+t1073+t164.*t620-t101.*t1067-t164.*t1070))./2.0)-qd2.*(t393+t400+t412+t422+t437+t443+t475+t848+t852+t862+t885+t909+t910+t973+t1418+t1459+t1531+t1553+t2200+t2201+t2202+t2203+(t148.*(t969+t970+t971+t972+t1501-t8.*t65.*2.269795582384779e-33-t13.*t139.*4.451823873129729e-33))./2.0-(t827.*(t1429+t121.*(t962+t964+t965+t966+t967+t1355-t8.*t837.*1.097689519141626e-1-t13.*t883.*2.152934142846781e-1).*5.515-t12.*t876.*5.515+t514.*t806.*5.515))./2.0+(t827.*(t887+t1379+t1380+t1381+t1382-t11.*t758.*1.917749226941314e-35+t13.*t758.*4.451823873129729e-33))./2.0-t31.*t120.*1.874699728327322e-33-t12.*t309.*1.874699728327322e-33-t15.*t321.*1.874699728327322e-33-(t15.*t388)./2.0-t95.*t366.*1.874699728327322e-33-t124.*t345.*1.874699728327322e-33-(t101.*t398)./2.0-(t129.*t456)./2.0-(t164.*t488)./2.0-(t148.*t847)./2.0-(t292.*t711)./2.0-(t111.*t905)./2.0-(t372.*t976)./2.0+(t829.*t1186)./2.0-(t878.*t1190)./2.0+(t977.*t1221)./2.0-(t1225.*t1405)./2.0-(t851.*(t1430-t12.*t978.*(3.49e2./2.0e2)+t453.*t806.*(3.49e2./2.0e2)+t121.*(t836+t914+t915+t916+t1358-t8.*t837.*1.4967e-2).*(3.49e2./2.0e2)))./2.0),-qd1.*(t393+t400+t412+t422+t437+t443+t475+t848+t852+t862+t885+t909+t910+t973+t1418+t1459+t1531+t1553+t1783+t1784+t1786+t1788+t1789-t1790-t1791-t1792+t1794-t1796+t1798+t1799-t31.*t120.*1.874699728327322e-33-(t15.*t388)./2.0-(t101.*t398)./2.0-(t129.*t456)./2.0-(t164.*t488)./2.0-(t292.*t711)./2.0-(t372.*t976)./2.0-(t111.*t1749)./2.0-(t148.*t1738)./2.0-(t878.*t1190)./2.0-(t827.*t1742)./2.0-(t851.*t1746)./2.0-(t1225.*t1405)./2.0)-qd3.*(t2087+t2096+t2113+t2118+t2119+t2136+t2140+t2148+t2149+t2164+t2369+t2389+t2390+(t57.*(t2124+t2125+t2134+t2135-t366.*t758.*3.749399456654644e-33-t242.*t1532.*3.749399456654644e-33-t57.*t2129+t727.*(t2130+t2131+t2132+t2133-t729.*t942+t758.*t948)))./2.0-t31.*t120.*7.02899814278107e-66-t12.*t309.*7.02899814278107e-66-t15.*t321.*7.02899814278107e-66-t95.*t366.*7.02899814278107e-66-t124.*t345.*7.02899814278107e-66-(t57.*t1894)./2.0-(t711.*t1400)./2.0-(t878.*t1478)./2.0-(t976.*t1557)./2.0-(t727.*t1850)./2.0-(t1405.*t1564)./2.0-(t1378.*t1746)./2.0-(t1415.*t1738)./2.0-(t1467.*t1749)./2.0-(t1474.*t1742)./2.0+(t1771.*t1774)./2.0+(t1776.*t1779)./2.0+(t727.*(t2154+t2155+t2156+t2157+t2158+t84.*t321.*3.749399456654644e-33-t242.*t1538.*3.749399456654644e-33-t57.*t2163))./2.0)-qd2.*(t393+t400+t412+t422+t437+t443+t475+t1914+t1917+t1920+t1921+t1922+t1923+t1927+t1929+t1930+t1932+t1933+t1934+t1935+t1936+t1937+t1938+t1941-t31.*t120.*3.749399456654644e-33-t12.*t309.*3.749399456654644e-33-t15.*t321.*3.749399456654644e-33-(t15.*t388)./2.0-t95.*t366.*3.749399456654644e-33-t124.*t345.*3.749399456654644e-33+t242.*t243.*3.749399456654644e-33-(t101.*t398)./2.0+t121.*t379.*3.749399456654644e-33-(t129.*t456)./2.0-(t164.*t488)./2.0+t57.*t1458+t727.*t961-t711.*t1488-t878.*t1390-t976.*t1507-t1405.*t1412-t1290.*t1742-t1305.*t1738+(t1186.*t1909)./2.0-t1349.*t1746-t1369.*t1749+t1424.*t1769+t1500.*t1779-t1623.*t1771+(t1498.*t1942)./2.0-t1694.*t1763)-qd4.*(t1062+t1085+t1086+t1087+t1106+t1112+t1823+t1828+t1908+t1955+t2580-t124.*t653.*1.874699728327322e-33-(t67.*t1036)./2.0-(t711.*t1580)./2.0-(t444.*t1850)./2.0+(t1060.*t1305)./2.0-(t1080.*t1305)./2.0-(t1115.*t1290)./2.0-(t878.*t1575)./2.0-(t878.*t1602)./2.0+(t711.*t1910)./2.0+(t714.*t1909)./2.0-(t1110.*t1514)./2.0-(t729.*t1897)./2.0-(t806.*t1894)./2.0-(t1290.*t1956)./2.0-(t1590.*t1738)./2.0-(t1500.*t1959)./2.0+(t1779.*t1855)./2.0-(t1771.*t1871)./2.0-(t1771.*t1875)./2.0+(t1806.*t1942)./2.0+(t12.*(t2573+t2574+t2575-t100.*t124.*3.749399456654644e-33+t727.*t1603))./2.0+(t121.*(t1921+t1922+t1923+t1930+t1933+t1934+t1941-t124.*t345.*3.749399456654644e-33))./2.0),qd1.*(t2060+t2364+t2368+t2372+t2396-(t727.*(t1039+t1040-t2238+t727.*(t1023+t1025+t1041+t1042-t1053-t1004.*t2233)+t57.*t2279-t727.*t2280-t57.*(t1026+t1027+t1043-t1049-t1050-t960.*t2233)))./2.0+(t57.*(t2281+t2282+t2296-t57.*t2280-t727.*t2279))./2.0+(t416.*t976)./2.0-(t177.*t2094)./2.0+(t57.*t2278)./2.0-(t57.*t2292)./2.0+(t111.*t2285)./2.0+(t993.*t1405)./2.0-(t983.*t1467)./2.0-(t57.*t2566)./2.0+(t878.*t1803)./2.0-(t1343.*t1378)./2.0-(t727.*t2275)./2.0-(t727.*t2313)./2.0+(t851.*t2245)./2.0+(t827.*t2271)./2.0-(t1474.*t1782)./2.0-(t1155.*t2106)./2.0+(t727.*t2557)./2.0-(t727.*t2563)./2.0-(t1227.*t2091)./2.0-(t2028.*t2302)./2.0-(t2103.*t2434)./2.0+(t57.*(-t1038+t2045+t2266+t2268+t2567-t727.*t2263-t57.*(t2264+t2265-t766.*t2248)))./2.0-(t57.*(-t2064+t2281+t2282+t2293+t2296-t727.*(t1026+t1027+t1043-t1049-t1050-t2295)-t57.*(t1023+t1025+t1041+t1042-t1053-t2294)))./2.0+(t2299.*(t403+t404+t405+t406-t833-t853))./2.0+(t2241.*(t140+t141+t142+t143+t144+t146+t147-t205+t2242-t13.*t2233.*2.152934142846781e-1))./2.0)-qd4.*(t2482+t2483+t2489+t2494+t2512+t2513+t2527-t124.*t653.*7.02899814278107e-66+t121.*t1084.*1.874699728327322e-33-(t57.*t2426)./2.0-(t57.*t2509)./2.0-(t1115.*t1474)./2.0+t444.*t2340.*1.874699728327322e-33-(t878.*t2180)./2.0+(t878.*t2199)./2.0+t806.*t2278.*1.874699728327322e-33-(t1110.*t2106)./2.0-(t1474.*t1956)./2.0+(t1911.*t2271)./2.0-(t2103.*t2411)./2.0+(t2241.*t2416)./2.0-(t2299.*t2412)./2.0+(t2302.*t2415)./2.0-(t2299.*t2435)./2.0-(t2343.*t2408)./2.0-(t2351.*t2404)./2.0+(t2363.*t2405)./2.0+(t2362.*t2407)./2.0-(t2302.*t2490)./2.0-(t2363.*t2452)./2.0-(t2343.*t2511)./2.0+(t727.*(t2427+t2429+t806.*t2324))./2.0+(t806.*(t2345+t2347+t2348+t2361-t488.*t766.*3.749399456654644e-33-t100.*t2038.*3.749399456654644e-33+t57.*t2358+t727.*t2360))./2.0-(t121.*(t2088+t2117+t2137-t101.*t398.*3.749399456654644e-33-t129.*t456.*3.749399456654644e-33-t164.*t488.*3.749399456654644e-33+t57.*t2278+t727.*t2340))./2.0-(t444.*(t2318+t2319+t2325+t134.*t2233.*3.749399456654644e-33+t57.*t2324-t442.*t2250.*3.749399456654644e-33-t488.*t2252.*3.749399456654644e-33+t727.*t2327))./2.0)+qd2.*(-t2087-t2096-t2118-t2119-t2136-t2140-t2148-t2149-t2164+t2364+t2368-t2369+t2372-t2384-t2389-t2390+t2396+t120.*(t29+t30).*7.02899814278107e-66+(t2299.*(t1460+t1461+t1462+t1463+t1464-t1872-t1873))./2.0-(t727.*(t2155+t2156+t2157+t2158-t242.*t1538.*3.749399456654644e-33-t321.*t2233.*3.749399456654644e-33-t57.*(t2159+t2160+t2161-t2399-t2400-t1445.*t2233)+t727.*(t2150+t2151+t2153-t2397-t2398-t935.*t2233)))./2.0+t12.*t309.*7.02899814278107e-66+t15.*t321.*7.02899814278107e-66+t95.*t366.*7.02899814278107e-66+t124.*t345.*7.02899814278107e-66-(t57.*t2292)./2.0+(t878.*t1478)./2.0+(t878.*t1514)./2.0+(t976.*t1493)./2.0+(t57.*t2417)./2.0+(t976.*t1557)./2.0+(t57.*t2597)./2.0-(t1378.*t1471)./2.0-(t1441.*t1467)./2.0+(t1405.*t1519)./2.0+(t1405.*t1564)./2.0-(t727.*t2275)./2.0-(t727.*t2313)./2.0+(t1378.*t1746)./2.0-t727.*t2470.*1.874699728327322e-33+(t1467.*t1749)./2.0+(t1474.*t1742)./2.0+(t727.*t2600)./2.0-(t1221.*t2106)./2.0-(t1474.*t1919)./2.0+(t1290.*t2271)./2.0-(t1495.*t2094)./2.0+(t1349.*t2245)./2.0-(t1521.*t2091)./2.0-(t1421.*t2205)./2.0+(t1369.*t2285)./2.0-(t1768.*t1916)./2.0+(t1424.*t2392)./2.0-(t1942.*t2363)./2.0-(t2165.*t2302)./2.0-(t2103.*t2458)./2.0+(t2241.*t2472)./2.0+(t2299.*t2446)./2.0-(t2362.*t2455)./2.0+(t2302.*t2572)./2.0+(t1913.*(t1760-t1939))./2.0+(t2481.*(t1866-t2373))./2.0+(t2601.*(t1962-t2374))./2.0+(t2453.*(t2206-t2365))./2.0+((t1926-t2084).*(t1962-t2374))./2.0)+qd3.*(t57.*(t2345+t2347+t2348+t2361+t57.*(t2346+t751.*t1127-t766.*t1136-t780.*t2038+t762.*t2208+t788.*t2209)+t727.*(t2349+t675.*t734-t762.*t1093-t764.*t2038+t673.*t2209-t751.*t2207)-t488.*t766.*3.749399456654644e-33-t100.*t2038.*3.749399456654644e-33).*(-1.0./2.0)-(t727.*(t120.*t139.*3.749399456654644e-33+t84.*t242.*3.749399456654644e-33-t84.*t388.*3.749399456654644e-33+t139.*t421.*3.749399456654644e-33-t436.*t444.*3.749399456654644e-33-t57.*(t84.*t1008-t139.*t1004-t84.*t2228+t139.*t2222+t444.*t2226)+t727.*(-t84.*t930+t139.*t960+t84.*t2219-t139.*t2212+t444.*t2216)))./2.0+t15.*t134.*7.02899814278107e-66+t95.*t120.*7.02899814278107e-66+t15.*t242.*7.02899814278107e-66-t15.*t388.*7.02899814278107e-66+t100.*t392.*7.02899814278107e-66-t101.*t398.*7.02899814278107e-66+t95.*t421.*7.02899814278107e-66+t121.*t436.*7.02899814278107e-66+t124.*t442.*7.02899814278107e-66-t129.*t456.*7.02899814278107e-66-t164.*t488.*7.02899814278107e-66+t727.*t1105.*1.874699728327322e-33+t57.*t2278.*1.874699728327322e-33+t57.*t2289.*1.874699728327322e-33+(t711.*t2103)./2.0+(t878.*t2106)./2.0-t727.*t2275.*1.874699728327322e-33+(t976.*t2094)./2.0+(t1405.*t2091)./2.0+(t1378.*t2245)./2.0+(t1415.*t2241)./2.0+(t1474.*t2271)./2.0+(t1467.*t2285)./2.0+(t1771.*t2351)./2.0+(t1776.*t2362)./2.0+(t57.*(t120.*t758.*3.749399456654644e-33-t242.*t734.*3.749399456654644e-33+t388.*t734.*3.749399456654644e-33+t421.*t758.*3.749399456654644e-33+t436.*t806.*3.749399456654644e-33+t57.*(t734.*t1008+t758.*t1004-t734.*t2228-t758.*t2222+t806.*t2226)-t727.*(-t734.*t930-t758.*t960+t734.*t2219+t806.*t2216+t2212.*(t750-t754))))./2.0+(t2205.*(t1760-t1939))./2.0+(t2392.*(t1765-t2111))./2.0+(t727.*(t2318+t2319+t2325-t442.*t775.*3.749399456654644e-33-t488.*t783.*3.749399456654644e-33-t134.*(t79-t85).*3.749399456654644e-33+t727.*(t2314+t2315+t2316+t2317+t673.*t2050-t646.*t2207)-t57.*(t84.*t772-t646.*t1127+t783.*t1136-t780.*t2054-t788.*t2050+t775.*t2208)))./2.0),-qd4.*(-t2694-t2695-t2698-t2703+t2712+t2716+t2717+t2729+t121.*t2728+t444.*t2526+t1115.*t1911-t806.*t2509-t878.*t2626+t2416.*t2490-t2407.*t2511+t2299.*t2636+t2363.*t2704-(t2411.*t2697)./2.0)+qd2.*(-t1062-t1085-t1086-t1087-t1112-t1823+t2568+t2587+t2602+t2603+t2673+t2674-t2678+t2681+t2682+t2683+t2685+t2690+t2691+t2692+(t1115.*t1290)./2.0+(t878.*t1602)./2.0-(t12.*t2677)./2.0-(t121.*t2687)./2.0-(t2299.*t2606)./2.0+(t2472.*t2490)./2.0+(t2455.*t2511)./2.0+(t2363.*t2689)./2.0-(t2458.*t2697)./2.0-(t1742.*(t1611-t2004))./2.0-(t2572.*(t1807-t2536))./2.0-(t2736.*(t1866-t2373))./2.0-(t444.*(t2120+t2121+t2123+t2312-t2375-t2376))./2.0-(t2299.*(t1640-t2005-t2006+t2598))./2.0)-qd1.*(t1062+t1085+t1086+t1087+t1112+t1823-t2568-t2569-t2570-t2587-t2648-t2650-t2652+t2678-(t805.*t878)./2.0-(t827.*t1115)./2.0+(t444.*t2313)./2.0+(t444.*t2563)./2.0+(t806.*t2566)./2.0+(t2299.*t2307)./2.0+(t2412.*t2434)./2.0-(t2490.*t2547)./2.0)+qd3.*(-t2482-t2483-t2489-t2494-t2512-t2513-t2527+t2653+t2654+t2655+t2656+t2662+t2663+t2664+t2672),qd4.*((t444.*t1144)./2.0-(t806.*t1140)./2.0+(t806.*t1149)./2.0-(t444.*t2024)./2.0)+qd3.*(t1061+t1062+t1085+t1086+t1087+t1106+t1112+t1823+t1828+t1908+t2022+t2027-(t727.*(t1077+t1145+t1146-t444.*t814+t806.*t831))./2.0-t124.*t653.*1.874699728327322e-33-(t57.*t1140)./2.0-(t148.*t1080)./2.0-(t593.*t711)./2.0-(t805.*t878)./2.0-(t827.*t1115)./2.0-(t977.*t1110)./2.0+(t714.*(t403+t404+t405+t406-t833-t853))./2.0-(t827.*(t1120+t1121-t751.*t823.*5.515-t101.*(t825+t826+t828-t995+t1122+t1123).*5.515))./2.0)-qd1.*(t654+t1150+t1160+t2546+t2548-(t124.*t129)./2.0-(t100.*t164)./2.0-(t101.*t598)./2.0-(t164.*t613)./2.0)-qd2.*(t654+t1199+t1206+t1581+t1630+t1983+t1985+t2642+t2645-(t827.*(t1634+t1635+t1636+t101.*(t964+t965+t966-t1222+t1291-t2.*t20.*2.540928714850161e-34-t3.*t727.*4.149651502162508e-18-t8.*t837.*6.776895191416263e-2).*5.515))./2.0-(t124.*t129)./2.0-(t100.*t164)./2.0-(t101.*t598)./2.0-(t164.*t613)./2.0-(t292.*t714)./2.0-(t67.*t1603)./2.0+(t148.*t1605)./2.0+(t593.*t1186)./2.0-(t729.*t1639)./2.0),qd3.*(t1062+t1085+t1086+t1087+t1106+t1112+t1823+t1828+t1908+t1955+t2167+t2172+t2176+t2181+t2190+t2191+t2192+(t714.*(t1460+t1461+t1462+t1463+t1464-t1872-t1873))./2.0-t124.*t653.*1.874699728327322e-33-t12.*t1205.*1.874699728327322e-33-t121.*t1198.*1.874699728327322e-33-t444.*t1216.*1.874699728327322e-33-t806.*t1183.*1.874699728327322e-33-(t711.*t1580)./2.0-(t1080.*t1305)./2.0-(t1115.*t1290)./2.0-(t878.*t1602)./2.0-(t1110.*t1478)./2.0-(t1110.*t1514)./2.0-(t1415.*t1610)./2.0-(t1290.*t1956)./2.0-(t1500.*t1959)./2.0-(t1774.*t1806)./2.0-(t1771.*t1875)./2.0+(t1806.*(t1804-t1943))./2.0+(t1305.*(t1059-t1898-t1899+t2303))./2.0)-qd1.*(t654+t1199+t1206+t1581+t1630+t1982+t1983+t1984+t1985+t1986-(t124.*t129)./2.0-(t100.*t164)./2.0-(t101.*t598)./2.0-(t164.*t613)./2.0-(t292.*t714)./2.0-(t67.*t1603)./2.0-(t729.*t1639)./2.0+(t1159.*t1305)./2.0-(t827.*t1974)./2.0)-qd2.*(t654+t2007+t2008+t2009+t2010+t2012+t2013+t2016+t2017+t2019+t2020-(t124.*t129)./2.0-(t100.*t164)./2.0-(t101.*t598)./2.0-(t164.*t613)./2.0-t67.*t1603-t714.*t1488-t729.*t1639+t1110.*t1390+t1305.*t1610-t1290.*t1974-t1623.*t1806-t1500.*t1967)+qd4.*((t67.*t1140)./2.0+(t729.*t1144)./2.0+(t444.*t1997)./2.0-(t714.*t1910)./2.0-(t1110.*t1575)./2.0+(t806.*t2003)./2.0-(t1590.*t1610)./2.0+(t1806.*t1871)./2.0+(t1855.*t1967)./2.0-(t1911.*t1974)./2.0-(t12.*(t2619+t2620+t444.*t1603))./2.0-(t121.*(t2008+t2010+t2017+t2020-t67.*t1603-t729.*t1639))./2.0),qd1.*(t1062+t1085+t1086+t1087+t1112+t2459+t2473+t2478+t2558-t124.*t653.*1.874699728327322e-33-(t57.*t2185)./2.0-(t57.*t2531)./2.0+(t57.*t2545)./2.0-(t1281.*t1474)./2.0-(t827.*t1956)./2.0-(t1110.*t1803)./2.0-(t829.*t2411)./2.0+(t727.*t2535)./2.0-(t727.*t2543)./2.0-(t1155.*t2180)./2.0-(t2434.*t2435)./2.0+(t2415.*t2547)./2.0)-qd4.*(t2694+t2695+t2698+t2703-(t121.*t2702)./2.0-(t444.*t2528)./2.0-(t1110.*t2199)./2.0-(t1911.*t1956)./2.0+(t2411.*t2412)./2.0)-qd2.*(-t1062-t1085-t1086-t1087-t1112-t2191-t2192-t2459-t2473-t2478+t2559+t2568+t2582+t2586+t2588+t2592+t2595+t12.*t1205.*1.874699728327322e-33+t121.*t1198.*1.874699728327322e-33+t806.*t1183.*1.874699728327322e-33+(t1110.*t1478)./2.0+(t1110.*t1514)./2.0-t67.*t2578.*1.874699728327322e-33-(t57.*t2623)./2.0+t444.*t2470.*1.874699728327322e-33+(t1290.*t1956)./2.0-(t727.*t2639)./2.0+(t1909.*t2411)./2.0+(t1942.*t2404)./2.0+(t2411.*t2446)./2.0+(t2408.*t2455)./2.0-(t2404.*t2481)./2.0-(t2415.*t2472)./2.0-(t2302.*t2591)./2.0+(t2302.*t2640)./2.0+(t2343.*t2611)./2.0)-qd3.*(-t2482-t2483-t2489-t2494-t2512-t2513-t2527+t2653+t2654+t2655+t2656+t2662+t2663+t2664+t2672-t121.*t1084.*3.749399456654644e-33+t57.*t2426-t444.*t2340.*3.749399456654644e-33+t1110.*t2106-t806.*t2417.*3.749399456654644e-33-t727.*t2528+t1474.*t1956+t2103.*t2411-t2302.*t2415+t2343.*t2408+t2351.*t2404),-qd3.*(t2694+t2695+t2698+t2703-t2712-t2716-t2717-t2729+t806.*t1822.*1.874699728327322e-33+t121.*t2632.*1.874699728327322e-33-(t57.*t2711)./2.0-(t121.*t2728)./2.0+t444.*t2488.*1.874699728327322e-33-(t444.*t2526)./2.0-(t1115.*t1911)./2.0+(t1110.*t2180)./2.0+(t806.*t2509)./2.0+(t727.*t2720)./2.0+(t878.*t2626)./2.0-(t1474.*t2715)./2.0+(t2411.*t2435)./2.0-(t2404.*t2452)./2.0-(t2416.*t2490)./2.0+(t2407.*t2511)./2.0-(t2299.*t2636)./2.0+(t2302.*t2732)./2.0-(t2363.*t2704)./2.0+(t2343.*t2730)./2.0+(t2411.*t2697)./2.0)-qd1.*(t2747-t2748+t2749-t2753+t2754+(t805.*t1110)./2.0-(t444.*t2477)./2.0+(t444.*t2543)./2.0-(t1281.*t1911)./2.0+(t806.*t2531)./2.0-(t827.*t2715)./2.0+(t1155.*t2626)./2.0-(t2307.*t2411)./2.0+(t2416.*t2539)./2.0-(t2434.*t2636)./2.0+(t2547.*t2732)./2.0)-qd4.*((t121.*(t2633+t806.*t1822+t444.*t2488))./2.0+(t444.*t2720)./2.0-(t806.*t2711)./2.0+(t1110.*t2626)./2.0+(t1911.*t2715)./2.0-(t2411.*t2636)./2.0+(t2404.*t2704)./2.0+(t2407.*t2730)./2.0-(t2416.*t2732)./2.0)-qd2.*(-t2734-t2742-t2743-t2744-t2745-t2746+t2747+t2749+t2754+(t1110.*t1575)./2.0+(t1110.*t1602)./2.0+(t12.*t2741)./2.0+(t121.*t2738)./2.0-(t444.*t2477)./2.0-(t1629.*t1911)./2.0+(t1221.*t2626)./2.0+(t1911.*t1974)./2.0-(t1290.*t2715)./2.0+(t2407.*t2594)./2.0+(t2416.*t2591)./2.0-(t2411.*t2606)./2.0+(t2407.*t2611)./2.0-(t2404.*t2689)./2.0-(t2458.*t2636)./2.0+(t2404.*t2736)./2.0-(t2453.*t2704)./2.0+(t2455.*t2730)./2.0+(t2472.*t2732)./2.0)],[4,4]);
